simulink library "ammclib_bam_S32K3xx"  (R2016a)
(part 24 of 50)

      |       tmpOutCnt=tmpOutCnt+1;
      |       set_param([gcb '/fltState_Out'], 'Port', num2str(tmpOutCnt));
      |     end
      | 
      |   autoCalcEn=get_param(gcb,'autoCalcEn');
      |   if strcmp(autoCalcEn,'on')
      |     set_param(gcb,'MaskEnables',{'on','on','off','on','on','on','on','on','on','on','on','on','on','on','on','on','on','on','on','on','on','on','on','on','on','on','on','on','on','on','on','off'});
      |   else
      |     set_param(gcb,'MaskEnables',{'on','on','off','on','on','off','off','off','off','off','off','off','off','off','off','off','off','on','on','on','on','on','on','on','on','on','on','on','on','on','on','off'});
      |   end
      | 
      |     if (posblk(4) - posblk(2)) > 275
      |       height = 275;
      |       set_param(gcb,'Position',[posblk(1), posblk(2), posblk(3), posblk(2)+height])
      |     end
      |   end
      | else
      |   % shown state variables
      |   if strcmp(get_param([gcb '/fltUmaxDivImax'], 'BlockType'), 'Ground')
      |     posblk = get_param(gcb, 'Position');
      | 
      |     pos = get_param([gcb, '/fltUmaxDivImax'], 'Position');
      |     orient = get_param([gcb, '/fltUmaxDivImax'], 'Orientation');
      |     delete_block([gcb, '/fltUmaxDivImax']);
      |     add_block('built-in/Inport', [gcb, '/fltUmaxDivImax'], 'Position', pos, 'Orientation', orient, 'OutDataTypeStr', 'single');
      | 
      |     pos = get_param([gcb, '/fltLambdaW'], 'Position');
      |     orient = get_param([gcb, '/fltLambdaW'], 'Orientation');
      |     delete_block([gcb, '/fltLambdaW']);
      |     add_block('built-in/Inport', [gcb, '/fltLambdaW'], 'Position', pos, 'Orientation', orient, 'OutDataTypeStr', 'single');
      | 
      |     pos = get_param([gcb, '/fltLambdaFW'], 'Position');
      |     orient = get_param([gcb, '/fltLambdaFW'], 'Orientation');
      |     delete_block([gcb, '/fltLambdaFW']);
      |     add_block('built-in/Inport', [gcb, '/fltLambdaFW'], 'Position', pos, 'Orientation', orient, 'OutDataTypeStr', 'single');
      | 
      |     pos = get_param([gcb, '/fltPropGainQ'], 'Position');
      |     orient = get_param([gcb, '/fltPropGainQ'], 'Orientation');
      |     delete_block([gcb, '/fltPropGainQ']);
      |     add_block('built-in/Inport', [gcb, '/fltPropGainQ'], 'Position', pos, 'Orientation', orient, 'OutDataTypeStr', 'single');
      | 
      |     pos = get_param([gcb, '/fltIntegGainQ'], 'Position');
      |     orient = get_param([gcb, '/fltIntegGainQ'], 'Orientation');
      |     delete_block([gcb, '/fltIntegGainQ']);
      |     add_block('built-in/Inport', [gcb, '/fltIntegGainQ'], 'Position', pos, 'Orientation', orient, 'OutDataTypeStr', 'single');
      | 
      |     pos = get_param([gcb, '/fltLowerLimitQ'], 'Position');
      |     orient = get_param([gcb, '/fltLowerLimitQ'], 'Orientation');
      |     delete_block([gcb, '/fltLowerLimitQ']);
      |     add_block('built-in/Inport', [gcb, '/fltLowerLimitQ'], 'Position', pos, 'Orientation', orient, 'OutDataTypeStr', 'single');
      | 
      |     pos = get_param([gcb, '/fltUpperLimitQ'], 'Position');
      |     orient = get_param([gcb, '/fltUpperLimitQ'], 'Orientation');
      |     delete_block([gcb, '/fltUpperLimitQ']);
      |     add_block('built-in/Inport', [gcb, '/fltUpperLimitQ'], 'Position', pos, 'Orientation', orient, 'OutDataTypeStr', 'single');
      | 
      |     pos = get_param([gcb, '/fltPropGainFW'], 'Position');
      |     orient = get_param([gcb, '/fltPropGainFW'], 'Orientation');
      |     delete_block([gcb, '/fltPropGainFW']);
      |     add_block('built-in/Inport', [gcb, '/fltPropGainFW'], 'Position', pos, 'Orientation', orient, 'OutDataTypeStr', 'single');
      | 
      |     pos = get_param([gcb, '/fltIntegGainFW'], 'Position');
      |     orient = get_param([gcb, '/fltIntegGainFW'], 'Orientation');
      |     delete_block([gcb, '/fltIntegGainFW']);
      |     add_block('built-in/Inport', [gcb, '/fltIntegGainFW'], 'Position', pos, 'Orientation', orient, 'OutDataTypeStr', 'single');
      | 
      |     pos = get_param([gcb, '/fltLowerLimitFW'], 'Position');
      |     orient = get_param([gcb, '/fltLowerLimitFW'], 'Orientation');
      |     delete_block([gcb, '/fltLowerLimitFW']);
      |     add_block('built-in/Inport', [gcb, '/fltLowerLimitFW'], 'Position', pos, 'Orientation', orient, 'OutDataTypeStr', 'single');
      | 
      |     pos = get_param([gcb, '/fltUpperLimitFW'], 'Position');
      |     orient = get_param([gcb, '/fltUpperLimitFW'], 'Orientation');
      |     delete_block([gcb, '/fltUpperLimitFW']);
      |     add_block('built-in/Inport', [gcb, '/fltUpperLimitFW'], 'Position', pos, 'Orientation', orient, 'OutDataTypeStr', 'single');
      | 
      |     pos = get_param([gcb, '/fltRampUp'], 'Position');
      |     orient = get_param([gcb, '/fltRampUp'], 'Orientation');
      |     delete_block([gcb, '/fltRampUp']);
      |     add_block('built-in/Inport', [gcb, '/fltRampUp'], 'Position', pos, 'Orientation', orient, 'OutDataTypeStr', 'single');
      | 
      |     pos = get_param([gcb, '/fltRampDown'], 'Position');
      |     orient = get_param([gcb, '/fltRampDown'], 'Orientation');
      |     delete_block([gcb, '/fltRampDown']);
      |     add_block('built-in/Inport', [gcb, '/fltRampDown'], 'Position', pos, 'Orientation', orient, 'OutDataTypeStr', 'single');
      | 
      |     pos = get_param([gcb, '/fltIQReqK_1'], 'Position');
      |     orient = get_param([gcb, '/fltIQReqK_1'], 'Orientation');
      |     delete_block([gcb, '/fltIQReqK_1']);
      |     add_block('built-in/Inport', [gcb, '/fltIQReqK_1'], 'Position', pos, 'Orientation', orient, 'OutDataTypeStr', 'single');
      | 
      |     pos = get_param([gcb, '/fltAccW'], 'Position');
      |     orient = get_param([gcb, '/fltAccW'], 'Orientation');
      |     delete_block([gcb, '/fltAccW']);
      |     add_block('built-in/Inport', [gcb, '/fltAccW'], 'Position', pos, 'Orientation', orient, 'OutDataTypeStr', 'single');
      | 
      |     pos = get_param([gcb, '/fltAccFW'], 'Position');
      |     orient = get_param([gcb, '/fltAccFW'], 'Orientation');
      |     delete_block([gcb, '/fltAccFW']);
      |     add_block('built-in/Inport', [gcb, '/fltAccFW'], 'Position', pos, 'Orientation', orient, 'OutDataTypeStr', 'single');
      | 
      |     pos = get_param([gcb, '/fltIntegPartK_1Q'], 'Position');
      |     orient = get_param([gcb, '/fltIntegPartK_1Q'], 'Orientation');
      |     delete_block([gcb, '/fltIntegPartK_1Q']);
      |     add_block('built-in/Inport', [gcb, '/fltIntegPartK_1Q'], 'Position', pos, 'Orientation', orient, 'OutDataTypeStr', 'single');
      | 
      |     pos = get_param([gcb, '/fltInK_1Q'], 'Position');
      |     orient = get_param([gcb, '/fltInK_1Q'], 'Orientation');
      |     delete_block([gcb, '/fltInK_1Q']);
      |     add_block('built-in/Inport', [gcb, '/fltInK_1Q'], 'Position', pos, 'Orientation', orient, 'OutDataTypeStr', 'single');
      | 
      |     pos = get_param([gcb, '/fltIntegPartK_1FW'], 'Position');
      |     orient = get_param([gcb, '/fltIntegPartK_1FW'], 'Orientation');
      |     delete_block([gcb, '/fltIntegPartK_1FW']);
      |     add_block('built-in/Inport', [gcb, '/fltIntegPartK_1FW'], 'Position', pos, 'Orientation', orient, 'OutDataTypeStr', 'single');
      | 
      |     pos = get_param([gcb, '/fltInK_1FW'], 'Position');
      |     orient = get_param([gcb, '/fltInK_1FW'], 'Orientation');
      |     delete_block([gcb, '/fltInK_1FW']);
      |     add_block('built-in/Inport', [gcb, '/fltInK_1FW'], 'Position', pos, 'Orientation', orient, 'OutDataTypeStr', 'single');
      | 
      |     pos = get_param([gcb, '/fltState'], 'Position');
      |     orient = get_param([gcb, '/fltState'], 'Orientation');
      |     delete_block([gcb, '/fltState']);
      |     add_block('built-in/Inport', [gcb, '/fltState'], 'Position', pos, 'Orientation', orient, 'OutDataTypeStr', 'single');
      | 
      | 
      | 
      |     pos = get_param([gcb '/fltAccW_Out'], 'Position');
      |     orient = get_param([gcb '/fltAccW_Out'], 'Orientation');
      |     delete_block([gcb '/fltAccW_Out']);
      |     add_block('built-in/Outport', [gcb '/fltAccW_Out'], 'Position', pos, 'Orientation', orient);
      | 
      |     pos = get_param([gcb '/fltAccFW_Out'], 'Position');
      |     orient = get_param([gcb '/fltAccFW_Out'], 'Orientation');
      |     delete_block([gcb '/fltAccFW_Out']);
      |     add_block('built-in/Outport', [gcb '/fltAccFW_Out'], 'Position', pos, 'Orientation', orient);
      | 
      |     pos = get_param([gcb '/fltIntegPartK_1Q_Out'], 'Position');
      |     orient = get_param([gcb '/fltIntegPartK_1Q_Out'], 'Orientation');
      |     delete_block([gcb '/fltIntegPartK_1Q_Out']);
      |     add_block('built-in/Outport', [gcb '/fltIntegPartK_1Q_Out'], 'Position', pos, 'Orientation', orient);
      | 
      |     pos = get_param([gcb '/fltInK_1Q_Out'], 'Position');
      |     orient = get_param([gcb '/fltInK_1Q_Out'], 'Orientation');
      |     delete_block([gcb '/fltInK_1Q_Out']);
      |     add_block('built-in/Outport', [gcb '/fltInK_1Q_Out'], 'Position', pos, 'Orientation', orient);
      | 
      |     pos = get_param([gcb '/fltIntegPartK_1FW_Out'], 'Position');
      |     orient = get_param([gcb '/fltIntegPartK_1FW_Out'], 'Orientation');
      |     delete_block([gcb '/fltIntegPartK_1FW_Out']);
      |     add_block('built-in/Outport', [gcb '/fltIntegPartK_1FW_Out'], 'Position', pos, 'Orientation', orient);
      | 
      |     pos = get_param([gcb '/fltInK_1FW_Out'], 'Position');
      |     orient = get_param([gcb '/fltInK_1FW_Out'], 'Orientation');
      |     delete_block([gcb '/fltInK_1FW_Out']);
      |     add_block('built-in/Outport', [gcb '/fltInK_1FW_Out'], 'Position', pos, 'Orientation', orient);
      | 
      | 
      |     pmask=Simulink.Mask.get(gcb);
      |     pctrl=pmask.getParameter('SampleTime');
      |     pctrl.set('TypeOptions',{'fltVelocityReq/SampleTime','fltVelocityFbck/SampleTime','fltIQFbck/SampleTime','fltUQReq/SampleTime','fltUQLim/SampleTime','fltFilterMAWOut_preset/SampleTime','fltFilterMAFWOut_preset/SampleTime','fltControllerPIpAWQOut_preset/SampleTime','fltControllerPIpAWFWOut_preset/SampleTime','fltRampOut_preset/SampleTime','fltUmaxDivImax/SampleTime','fltLambdaW/SampleTime','fltLambdaFW/SampleTime','fltPropGainQ/SampleTime','fltIntegGainQ/SampleTime','fltLowerLimitQ/SampleTime','fltUpperLimitQ/SampleTime','fltPropGainFW/SampleTime','fltIntegGainFW/SampleTime','fltLowerLimitFW/SampleTime','fltUpperLimitFW/SampleTime','fltRampUp/SampleTime','fltRampDown/SampleTime','fltIQReqK_1/SampleTime','fltAccW/SampleTime','fltAccFW/SampleTime','fltIntegPartK_1Q/SampleTime','fltInK_1Q/SampleTime','fltIntegPartK_1FW/SampleTime','fltInK_1FW/SampleTime','fltState/SampleTime'});
      | 
      |     if (showDebugOutputs == 2) && (strcmp(get_param([gcb '/fltWReqFilt'], 'BlockType'), 'Terminator'))
      |       pos = get_param([gcb '/fltWReqFilt'], 'Position');
      |       orient = get_param([gcb '/fltWReqFilt'], 'Orientation');
      |       delete_block([gcb '/fltWReqFilt']);
      |       add_block('built-in/Outport', [gcb '/fltWReqFilt'], 'Position', pos, 'Orientation', orient);
      | 
      |       pos = get_param([gcb '/fltWErr'], 'Position');
      |       orient = get_param([gcb '/fltWErr'], 'Orientation');
      |       delete_block([gcb '/fltWErr']);
      |       add_block('built-in/Outport', [gcb '/fltWErr'], 'Position', pos, 'Orientation', orient);
      | 
      |       pos = get_param([gcb '/fltIDQReqAmp'], 'Position');
      |       orient = get_param([gcb '/fltIDQReqAmp'], 'Orientation');
      |       delete_block([gcb '/fltIDQReqAmp']);
      |       add_block('built-in/Outport', [gcb '/fltIDQReqAmp'], 'Position', pos, 'Orientation', orient);
      | 
      |       pos = get_param([gcb '/fltWFbckFilt'], 'Position');
      |       orient = get_param([gcb '/fltWFbckFilt'], 'Orientation');
      |       delete_block([gcb '/fltWFbckFilt']);
      |       add_block('built-in/Outport', [gcb '/fltWFbckFilt'], 'Position', pos, 'Orientation', orient);
      | 
      |       pos = get_param([gcb '/fltIQErrSign'], 'Position');
      |       orient = get_param([gcb '/fltIQErrSign'], 'Orientation');
      |       delete_block([gcb '/fltIQErrSign']);
      |       add_block('built-in/Outport', [gcb '/fltIQErrSign'], 'Position', pos, 'Orientation', orient);
      | 
      |       pos = get_param([gcb '/fltFWErr'], 'Position');
      |       orient = get_param([gcb '/fltFWErr'], 'Orientation');
      |       delete_block([gcb '/fltFWErr']);
      |       add_block('built-in/Outport', [gcb '/fltFWErr'], 'Position', pos, 'Orientation', orient);
      | 
      |       pos = get_param([gcb '/fltIQErr'], 'Position');
      |       orient = get_param([gcb '/fltIQErr'], 'Orientation');
      |       delete_block([gcb '/fltIQErr']);
      |       add_block('built-in/Outport', [gcb '/fltIQErr'], 'Position', pos, 'Orientation', orient);
      | 
      |       pos = get_param([gcb '/fltUQErr'], 'Position');
      |       orient = get_param([gcb '/fltUQErr'], 'Orientation');
      |       delete_block([gcb '/fltUQErr']);
      |       add_block('built-in/Outport', [gcb '/fltUQErr'], 'Position', pos, 'Orientation', orient);
      | 
      |       pos = get_param([gcb '/fltFWErrFilt'], 'Position');
      |       orient = get_param([gcb '/fltFWErrFilt'], 'Orientation');
      |       delete_block([gcb '/fltFWErrFilt']);
      |       add_block('built-in/Outport', [gcb '/fltFWErrFilt'], 'Position', pos, 'Orientation', orient);
      | 
      |       pos = get_param([gcb '/fltFWAngle'], 'Position');
      |       orient = get_param([gcb '/fltFWAngle'], 'Orientation');
      |       delete_block([gcb '/fltFWAngle']);
      |       add_block('built-in/Outport', [gcb '/fltFWAngle'], 'Position', pos, 'Orientation', orient);
      | 
      |       pos = get_param([gcb '/fltFWSin'], 'Position');
      |       orient = get_param([gcb '/fltFWSin'], 'Orientation');
      |       delete_block([gcb '/fltFWSin']);
      |       add_block('built-in/Outport', [gcb '/fltFWSin'], 'Position', pos, 'Orientation', orient);
      | 
      |       pos = get_param([gcb '/fltFWCos'], 'Position');
      |       orient = get_param([gcb '/fltFWCos'], 'Orientation');
      |       delete_block([gcb '/fltFWCos']);
      |       add_block('built-in/Outport', [gcb '/fltFWCos'], 'Position', pos, 'Orientation', orient);
      | 
      |     end
      | 
      |     set_param([gcb '/fltVelocityReq'], 'Port', '1');
      |     set_param([gcb '/fltVelocityFbck'], 'Port', '2');
      |     set_param([gcb '/fltIQFbck'], 'Port', '3');
      |     set_param([gcb '/fltUQReq'], 'Port', '4');
      |     set_param([gcb '/fltUQLim'], 'Port', '5');
      |     set_param([gcb '/fltFilterMAWOut_preset'], 'Port', '6');
      |     set_param([gcb '/fltFilterMAFWOut_preset'], 'Port', '7');
      |     set_param([gcb '/fltControllerPIpAWQOut_preset'], 'Port', '8');
      |     set_param([gcb '/fltControllerPIpAWFWOut_preset'], 'Port', '9');
      |     set_param([gcb '/fltRampOut_preset'], 'Port', '10');
      |     set_param([gcb '/fltUmaxDivImax'], 'Port', '11');
      |     set_param([gcb '/fltLambdaW'], 'Port', '12');
      |     set_param([gcb '/fltLambdaFW'], 'Port', '13');
      |     set_param([gcb '/fltPropGainQ'], 'Port', '14');
      |     set_param([gcb '/fltIntegGainQ'], 'Port', '15');
      |     set_param([gcb '/fltLowerLimitQ'], 'Port', '16');
      |     set_param([gcb '/fltUpperLimitQ'], 'Port', '17');
      |     set_param([gcb '/fltPropGainFW'], 'Port', '18');
      |     set_param([gcb '/fltIntegGainFW'], 'Port', '19');
      |     set_param([gcb '/fltLowerLimitFW'], 'Port', '20');
      |     set_param([gcb '/fltUpperLimitFW'], 'Port', '21');
      |     set_param([gcb '/fltRampUp'], 'Port', '22');
      |     set_param([gcb '/fltRampDown'], 'Port', '23');
      |     set_param([gcb '/fltIQReqK_1'], 'Port', '24');
      |     set_param([gcb '/fltAccW'], 'Port', '25');
      |     set_param([gcb '/fltAccFW'], 'Port', '26');
      |     set_param([gcb '/fltIntegPartK_1Q'], 'Port', '27');
      |     set_param([gcb '/fltInK_1Q'], 'Port', '28');
      |     set_param([gcb '/fltIntegPartK_1FW'], 'Port', '29');
      |     set_param([gcb '/fltInK_1FW'], 'Port', '30');
      |     set_param([gcb '/fltState'], 'Port', '31');
      | 
      |     if (showDebugOutputs == 2)
      |       tmpOutCnt=0;
      |       tmpOutCnt=tmpOutCnt+1;
      |       set_param([gcb '/pIDQReq'], 'Port', num2str(tmpOutCnt));
      |       tmpOutCnt=tmpOutCnt+1;
      |       set_param([gcb '/u16LimitFlagQ'], 'Port', num2str(tmpOutCnt));
      |       tmpOutCnt=tmpOutCnt+1;
      |       set_param([gcb '/u16LimitFlagFW'], 'Port', num2str(tmpOutCnt));
      |       tmpOutCnt=tmpOutCnt+1;
      |       set_param([gcb '/fltWReqFilt'], 'Port', num2str(tmpOutCnt));
      |       tmpOutCnt=tmpOutCnt+1;
      |       set_param([gcb '/fltWErr'], 'Port', num2str(tmpOutCnt));
      |       tmpOutCnt=tmpOutCnt+1;
      |       set_param([gcb '/fltIDQReqAmp'], 'Port', num2str(tmpOutCnt));
      |       tmpOutCnt=tmpOutCnt+1;
      |       set_param([gcb '/fltWFbckFilt'], 'Port', num2str(tmpOutCnt));
      |       tmpOutCnt=tmpOutCnt+1;
      |       set_param([gcb '/fltIQErrSign'], 'Port', num2str(tmpOutCnt));
      |       tmpOutCnt=tmpOutCnt+1;
      |       set_param([gcb '/fltFWErr'], 'Port', num2str(tmpOutCnt));
      |       tmpOutCnt=tmpOutCnt+1;
      |       set_param([gcb '/fltIQErr'], 'Port', num2str(tmpOutCnt));
      |       tmpOutCnt=tmpOutCnt+1;
      |       set_param([gcb '/fltUQErr'], 'Port', num2str(tmpOutCnt));
      |       tmpOutCnt=tmpOutCnt+1;
      |       set_param([gcb '/fltFWErrFilt'], 'Port', num2str(tmpOutCnt));
      |       tmpOutCnt=tmpOutCnt+1;
      |       set_param([gcb '/fltFWAngle'], 'Port', num2str(tmpOutCnt));
      |       tmpOutCnt=tmpOutCnt+1;
      |       set_param([gcb '/fltFWSin'], 'Port', num2str(tmpOutCnt));
      |       tmpOutCnt=tmpOutCnt+1;
      |       set_param([gcb '/fltFWCos'], 'Port', num2str(tmpOutCnt));
      |       tmpOutCnt=tmpOutCnt+1;
      |       set_param([gcb '/fltAccW_Out'], 'Port', num2str(tmpOutCnt));
      |       tmpOutCnt=tmpOutCnt+1;
      |       set_param([gcb '/fltAccFW_Out'], 'Port', num2str(tmpOutCnt));
      |       tmpOutCnt=tmpOutCnt+1;
      |       set_param([gcb '/fltIntegPartK_1Q_Out'], 'Port', num2str(tmpOutCnt));
      |       tmpOutCnt=tmpOutCnt+1;
      |       set_param([gcb '/fltInK_1Q_Out'], 'Port', num2str(tmpOutCnt));
      |       tmpOutCnt=tmpOutCnt+1;
      |       set_param([gcb '/fltIntegPartK_1FW_Out'], 'Port', num2str(tmpOutCnt));
      |       tmpOutCnt=tmpOutCnt+1;
      |       set_param([gcb '/fltInK_1FW_Out'], 'Port', num2str(tmpOutCnt));
      |       if strcmp(get_param([gcb '/fltState_Out'], 'BlockType'), 'Outport')
      |         tmpOutCnt=tmpOutCnt+1;
      |         set_param([gcb '/fltState_Out'], 'Port', num2str(tmpOutCnt));
      |       end
      |     else
      |       tmpOutCnt=0;
      |       tmpOutCnt=tmpOutCnt+1;
      |       set_param([gcb '/pIDQReq'], 'Port', num2str(tmpOutCnt));
      |       tmpOutCnt=tmpOutCnt+1;
      |       set_param([gcb '/u16LimitFlagQ'], 'Port', num2str(tmpOutCnt));
      |       tmpOutCnt=tmpOutCnt+1;
      |       set_param([gcb '/u16LimitFlagFW'], 'Port', num2str(tmpOutCnt));
      |       tmpOutCnt=tmpOutCnt+1;
      |       set_param([gcb '/fltAccW_Out'], 'Port', num2str(tmpOutCnt));
      |       tmpOutCnt=tmpOutCnt+1;
      |       set_param([gcb '/fltAccFW_Out'], 'Port', num2str(tmpOutCnt));
      |       tmpOutCnt=tmpOutCnt+1;
      |       set_param([gcb '/fltIntegPartK_1Q_Out'], 'Port', num2str(tmpOutCnt));
      |       tmpOutCnt=tmpOutCnt+1;
      |       set_param([gcb '/fltInK_1Q_Out'], 'Port', num2str(tmpOutCnt));
      |       tmpOutCnt=tmpOutCnt+1;
      |       set_param([gcb '/fltIntegPartK_1FW_Out'], 'Port', num2str(tmpOutCnt));
      |       tmpOutCnt=tmpOutCnt+1;
      |       set_param([gcb '/fltInK_1FW_Out'], 'Port', num2str(tmpOutCnt));
      |       if strcmp(get_param([gcb '/fltState_Out'], 'BlockType'), 'Outport')
      |         tmpOutCnt=tmpOutCnt+1;
      |         set_param([gcb '/fltState_Out'], 'Port', num2str(tmpOutCnt));
      |       end
      |     end
      | 
      |     set_param(gcb,'MaskEnables',{'on','on','on','on','on','off','off','off','off','off','off','off','off','off','off','off','off','off','off','off','off','off','off','off','off','off','off','off','off','off','off','off'});
      | 
      |     if (posblk(4) - posblk(2)) < 800
      |       height = 800;
      |       set_param(gcb,'Position',[posblk(1), posblk(2), posblk(3), posblk(2)+height])
      |     end
      |   else
      |     if (showDebugOutputs == 2) && (strcmp(get_param([gcb '/fltWReqFilt'], 'BlockType'), 'Terminator'))
      |       % shown debugging outputs
      |       pos = get_param([gcb '/fltWReqFilt'], 'Position');
      |       orient = get_param([gcb '/fltWReqFilt'], 'Orientation');
      |       delete_block([gcb '/fltWReqFilt']);
      |       add_block('built-in/Outport', [gcb '/fltWReqFilt'], 'Position', pos, 'Orientation', orient);
      | 
      |       pos = get_param([gcb '/fltWErr'], 'Position');
      |       orient = get_param([gcb '/fltWErr'], 'Orientation');
      |       delete_block([gcb '/fltWErr']);
      |       add_block('built-in/Outport', [gcb '/fltWErr'], 'Position', pos, 'Orientation', orient);
      | 
      |       pos = get_param([gcb '/fltIDQReqAmp'], 'Position');
      |       orient = get_param([gcb '/fltIDQReqAmp'], 'Orientation');
      |       delete_block([gcb '/fltIDQReqAmp']);
      |       add_block('built-in/Outport', [gcb '/fltIDQReqAmp'], 'Position', pos, 'Orientation', orient);
      | 
      |       pos = get_param([gcb '/fltWFbckFilt'], 'Position');
      |       orient = get_param([gcb '/fltWFbckFilt'], 'Orientation');
      |       delete_block([gcb '/fltWFbckFilt']);
      |       add_block('built-in/Outport', [gcb '/fltWFbckFilt'], 'Position', pos, 'Orientation', orient);
      | 
      |       pos = get_param([gcb '/fltIQErrSign'], 'Position');
      |       orient = get_param([gcb '/fltIQErrSign'], 'Orientation');
      |       delete_block([gcb '/fltIQErrSign']);
      |       add_block('built-in/Outport', [gcb '/fltIQErrSign'], 'Position', pos, 'Orientation', orient);
      | 
      |       pos = get_param([gcb '/fltFWErr'], 'Position');
      |       orient = get_param([gcb '/fltFWErr'], 'Orientation');
      |       delete_block([gcb '/fltFWErr']);
      |       add_block('built-in/Outport', [gcb '/fltFWErr'], 'Position', pos, 'Orientation', orient);
      | 
      |       pos = get_param([gcb '/fltIQErr'], 'Position');
      |       orient = get_param([gcb '/fltIQErr'], 'Orientation');
      |       delete_block([gcb '/fltIQErr']);
      |       add_block('built-in/Outport', [gcb '/fltIQErr'], 'Position', pos, 'Orientation', orient);
      | 
      |       pos = get_param([gcb '/fltUQErr'], 'Position');
      |       orient = get_param([gcb '/fltUQErr'], 'Orientation');
      |       delete_block([gcb '/fltUQErr']);
      |       add_block('built-in/Outport', [gcb '/fltUQErr'], 'Position', pos, 'Orientation', orient);
      | 
      |       pos = get_param([gcb '/fltFWErrFilt'], 'Position');
      |       orient = get_param([gcb '/fltFWErrFilt'], 'Orientation');
      |       delete_block([gcb '/fltFWErrFilt']);
      |       add_block('built-in/Outport', [gcb '/fltFWErrFilt'], 'Position', pos, 'Orientation', orient);
      | 
      |       pos = get_param([gcb '/fltFWAngle'], 'Position');
      |       orient = get_param([gcb '/fltFWAngle'], 'Orientation');
      |       delete_block([gcb '/fltFWAngle']);
      |       add_block('built-in/Outport', [gcb '/fltFWAngle'], 'Position', pos, 'Orientation', orient);
      | 
      |       pos = get_param([gcb '/fltFWSin'], 'Position');
      |       orient = get_param([gcb '/fltFWSin'], 'Orientation');
      |       delete_block([gcb '/fltFWSin']);
      |       add_block('built-in/Outport', [gcb '/fltFWSin'], 'Position', pos, 'Orientation', orient);
      | 
      |       pos = get_param([gcb '/fltFWCos'], 'Position');
      |       orient = get_param([gcb '/fltFWCos'], 'Orientation');
      |       delete_block([gcb '/fltFWCos']);
      |       add_block('built-in/Outport', [gcb '/fltFWCos'], 'Position', pos, 'Orientation', orient);
      | 
      |       tmpOutCnt=0;
      |       tmpOutCnt=tmpOutCnt+1;
      |       set_param([gcb '/pIDQReq'], 'Port', num2str(tmpOutCnt));
      |       tmpOutCnt=tmpOutCnt+1;
      |       set_param([gcb '/u16LimitFlagQ'], 'Port', num2str(tmpOutCnt));
      |       tmpOutCnt=tmpOutCnt+1;
      |       set_param([gcb '/u16LimitFlagFW'], 'Port', num2str(tmpOutCnt));
      |       tmpOutCnt=tmpOutCnt+1;
      |       set_param([gcb '/fltWReqFilt'], 'Port', num2str(tmpOutCnt));
      |       tmpOutCnt=tmpOutCnt+1;
      |       set_param([gcb '/fltWErr'], 'Port', num2str(tmpOutCnt));
      |       tmpOutCnt=tmpOutCnt+1;
      |       set_param([gcb '/fltIDQReqAmp'], 'Port', num2str(tmpOutCnt));
      |       tmpOutCnt=tmpOutCnt+1;
      |       set_param([gcb '/fltWFbckFilt'], 'Port', num2str(tmpOutCnt));
      |       tmpOutCnt=tmpOutCnt+1;
      |       set_param([gcb '/fltIQErrSign'], 'Port', num2str(tmpOutCnt));
      |       tmpOutCnt=tmpOutCnt+1;
      |       set_param([gcb '/fltFWErr'], 'Port', num2str(tmpOutCnt));
      |       tmpOutCnt=tmpOutCnt+1;
      |       set_param([gcb '/fltIQErr'], 'Port', num2str(tmpOutCnt));
      |       tmpOutCnt=tmpOutCnt+1;
      |       set_param([gcb '/fltUQErr'], 'Port', num2str(tmpOutCnt));
      |       tmpOutCnt=tmpOutCnt+1;
      |       set_param([gcb '/fltFWErrFilt'], 'Port', num2str(tmpOutCnt));
      |       tmpOutCnt=tmpOutCnt+1;
      |       set_param([gcb '/fltFWAngle'], 'Port', num2str(tmpOutCnt));
      |       tmpOutCnt=tmpOutCnt+1;
      |       set_param([gcb '/fltFWSin'], 'Port', num2str(tmpOutCnt));
      |       tmpOutCnt=tmpOutCnt+1;
      |       set_param([gcb '/fltFWCos'], 'Port', num2str(tmpOutCnt));
      |       tmpOutCnt=tmpOutCnt+1;
      |       set_param([gcb '/fltAccW_Out'], 'Port', num2str(tmpOutCnt));
      |       tmpOutCnt=tmpOutCnt+1;
      |       set_param([gcb '/fltAccFW_Out'], 'Port', num2str(tmpOutCnt));
      |       tmpOutCnt=tmpOutCnt+1;
      |       set_param([gcb '/fltIntegPartK_1Q_Out'], 'Port', num2str(tmpOutCnt));
      |       tmpOutCnt=tmpOutCnt+1;
      |       set_param([gcb '/fltInK_1Q_Out'], 'Port', num2str(tmpOutCnt));
      |       tmpOutCnt=tmpOutCnt+1;
      |       set_param([gcb '/fltIntegPartK_1FW_Out'], 'Port', num2str(tmpOutCnt));
      |       tmpOutCnt=tmpOutCnt+1;
      |       set_param([gcb '/fltInK_1FW_Out'], 'Port', num2str(tmpOutCnt));
      |       if strcmp(get_param([gcb '/fltState_Out'], 'BlockType'), 'Outport')
      |         tmpOutCnt=tmpOutCnt+1;
      |         set_param([gcb '/fltState_Out'], 'Port', num2str(tmpOutCnt));
      |       end
      |     elseif (showDebugOutputs == 1) && (strcmp(get_param([gcb '/fltWReqFilt'], 'BlockType'), 'Outport'))
      |       % hidden debugging outputs
      |       pos = get_param([gcb '/fltWReqFilt'], 'Position');
      |       orient = get_param([gcb '/fltWReqFilt'], 'Orientation');
      |       delete_block([gcb '/fltWReqFilt']);
      |       add_block('built-in/Terminator', [gcb '/fltWReqFilt'], 'Position', pos, 'Orientation', orient);
      | 
      |       pos = get_param([gcb '/fltWErr'], 'Position');
      |       orient = get_param([gcb '/fltWErr'], 'Orientation');
      |       delete_block([gcb '/fltWErr']);
      |       add_block('built-in/Terminator', [gcb '/fltWErr'], 'Position', pos, 'Orientation', orient);
      | 
      |       pos = get_param([gcb '/fltIDQReqAmp'], 'Position');
      |       orient = get_param([gcb '/fltIDQReqAmp'], 'Orientation');
      |       delete_block([gcb '/fltIDQReqAmp']);
      |       add_block('built-in/Terminator', [gcb '/fltIDQReqAmp'], 'Position', pos, 'Orientation', orient);
      | 
      |       pos = get_param([gcb '/fltWFbckFilt'], 'Position');
      |       orient = get_param([gcb '/fltWFbckFilt'], 'Orientation');
      |       delete_block([gcb '/fltWFbckFilt']);
      |       add_block('built-in/Terminator', [gcb '/fltWFbckFilt'], 'Position', pos, 'Orientation', orient);
      | 
      |       pos = get_param([gcb '/fltIQErrSign'], 'Position');
      |       orient = get_param([gcb '/fltIQErrSign'], 'Orientation');
      |       delete_block([gcb '/fltIQErrSign']);
      |       add_block('built-in/Terminator', [gcb '/fltIQErrSign'], 'Position', pos, 'Orientation', orient);
      | 
      |       pos = get_param([gcb '/fltFWErr'], 'Position');
      |       orient = get_param([gcb '/fltFWErr'], 'Orientation');
      |       delete_block([gcb '/fltFWErr']);
      |       add_block('built-in/Terminator', [gcb '/fltFWErr'], 'Position', pos, 'Orientation', orient);
      | 
      |       pos = get_param([gcb '/fltIQErr'], 'Position');
      |       orient = get_param([gcb '/fltIQErr'], 'Orientation');
      |       delete_block([gcb '/fltIQErr']);
      |       add_block('built-in/Terminator', [gcb '/fltIQErr'], 'Position', pos, 'Orientation', orient);
      | 
      |       pos = get_param([gcb '/fltUQErr'], 'Position');
      |       orient = get_param([gcb '/fltUQErr'], 'Orientation');
      |       delete_block([gcb '/fltUQErr']);
      |       add_block('built-in/Terminator', [gcb '/fltUQErr'], 'Position', pos, 'Orientation', orient);
      | 
      |       pos = get_param([gcb '/fltFWErrFilt'], 'Position');
      |       orient = get_param([gcb '/fltFWErrFilt'], 'Orientation');
      |       delete_block([gcb '/fltFWErrFilt']);
      |       add_block('built-in/Terminator', [gcb '/fltFWErrFilt'], 'Position', pos, 'Orientation', orient);
      | 
      |       pos = get_param([gcb '/fltFWAngle'], 'Position');
      |       orient = get_param([gcb '/fltFWAngle'], 'Orientation');
      |       delete_block([gcb '/fltFWAngle']);
      |       add_block('built-in/Terminator', [gcb '/fltFWAngle'], 'Position', pos, 'Orientation', orient);
      | 
      |       pos = get_param([gcb '/fltFWSin'], 'Position');
      |       orient = get_param([gcb '/fltFWSin'], 'Orientation');
      |       delete_block([gcb '/fltFWSin']);
      |       add_block('built-in/Terminator', [gcb '/fltFWSin'], 'Position', pos, 'Orientation', orient);
      | 
      |       pos = get_param([gcb '/fltFWCos'], 'Position');
      |       orient = get_param([gcb '/fltFWCos'], 'Orientation');
      |       delete_block([gcb '/fltFWCos']);
      |       add_block('built-in/Terminator', [gcb '/fltFWCos'], 'Position', pos, 'Orientation', orient);
      | 
      |       tmpOutCnt=0;
      |       tmpOutCnt=tmpOutCnt+1;
      |       set_param([gcb '/pIDQReq'], 'Port', num2str(tmpOutCnt));
      |       tmpOutCnt=tmpOutCnt+1;
      |       set_param([gcb '/u16LimitFlagQ'], 'Port', num2str(tmpOutCnt));
      |       tmpOutCnt=tmpOutCnt+1;
      |       set_param([gcb '/u16LimitFlagFW'], 'Port', num2str(tmpOutCnt));
      |       tmpOutCnt=tmpOutCnt+1;
      |       set_param([gcb '/fltAccW_Out'], 'Port', num2str(tmpOutCnt));
      |       tmpOutCnt=tmpOutCnt+1;
      |       set_param([gcb '/fltAccFW_Out'], 'Port', num2str(tmpOutCnt));
      |       tmpOutCnt=tmpOutCnt+1;
      |       set_param([gcb '/fltIntegPartK_1Q_Out'], 'Port', num2str(tmpOutCnt));
      |       tmpOutCnt=tmpOutCnt+1;
      |       set_param([gcb '/fltInK_1Q_Out'], 'Port', num2str(tmpOutCnt));
      |       tmpOutCnt=tmpOutCnt+1;
      |       set_param([gcb '/fltIntegPartK_1FW_Out'], 'Port', num2str(tmpOutCnt));
      |       tmpOutCnt=tmpOutCnt+1;
      |       set_param([gcb '/fltInK_1FW_Out'], 'Port', num2str(tmpOutCnt));
      |       if strcmp(get_param([gcb '/fltState_Out'], 'BlockType'), 'Outport')
      |         tmpOutCnt=tmpOutCnt+1;
      |         set_param([gcb '/fltState_Out'], 'Port', num2str(tmpOutCnt));
      |       end
      |     end
      |   end
      | end
      | if strcmp(get_param(gcb,'fltState_Out_showOutput'),'on')
      |   if strcmp(get_param([gcb '/fltState_Out'], 'BlockType'), 'Terminator')
      |     pos = get_param([gcb '/fltState_Out'], 'Position');
      |     orient = get_param([gcb '/fltState_Out'], 'Orientation');
      |     delete_block([gcb '/fltState_Out']);
      |     add_block('built-in/Outport', [gcb '/fltState_Out'], 'Position', pos, 'Orientation', orient);
      |     outputsChanged = 1;
      |   end
      | else
      |   if strcmp(get_param([gcb '/fltState_Out'], 'BlockType'), 'Outport')
      |     pos = get_param([gcb '/fltState_Out'], 'Position');
      |     orient = get_param([gcb '/fltState_Out'], 'Orientation');
      |     delete_block([gcb '/fltState_Out']);
      |     add_block('built-in/Terminator', [gcb '/fltState_Out'], 'Position', pos, 'Orientation', orient);
      |     outputsChanged = 1;
      |   end
      | end
      | if outputsChanged == 1;
      |   tmpOutCnt = 0;
      |   if strcmp(get_param([gcb '/pIDQReq'], 'BlockType'), 'Outport')
      |     tmpOutCnt = tmpOutCnt + 1;
      |     set_param([gcb '/pIDQReq'], 'Port', num2str(tmpOutCnt));
      |   end
      |   if strcmp(get_param([gcb '/u16LimitFlagQ'], 'BlockType'), 'Outport')
      |     tmpOutCnt = tmpOutCnt + 1;
      |     set_param([gcb '/u16LimitFlagQ'], 'Port', num2str(tmpOutCnt));
      |   end
      |   if strcmp(get_param([gcb '/u16LimitFlagFW'], 'BlockType'), 'Outport')
      |     tmpOutCnt = tmpOutCnt + 1;
      |     set_param([gcb '/u16LimitFlagFW'], 'Port', num2str(tmpOutCnt));
      |   end
      |   if strcmp(get_param([gcb '/fltWReqFilt'], 'BlockType'), 'Outport')
      |     tmpOutCnt = tmpOutCnt + 1;
      |     set_param([gcb '/fltWReqFilt'], 'Port', num2str(tmpOutCnt));
      |   end
      |   if strcmp(get_param([gcb '/fltWErr'], 'BlockType'), 'Outport')
      |     tmpOutCnt = tmpOutCnt + 1;
      |     set_param([gcb '/fltWErr'], 'Port', num2str(tmpOutCnt));
      |   end
      |   if strcmp(get_param([gcb '/fltIDQReqAmp'], 'BlockType'), 'Outport')
      |     tmpOutCnt = tmpOutCnt + 1;
      |     set_param([gcb '/fltIDQReqAmp'], 'Port', num2str(tmpOutCnt));
      |   end
      |   if strcmp(get_param([gcb '/fltWFbckFilt'], 'BlockType'), 'Outport')
      |     tmpOutCnt = tmpOutCnt + 1;
      |     set_param([gcb '/fltWFbckFilt'], 'Port', num2str(tmpOutCnt));
      |   end
      |   if strcmp(get_param([gcb '/fltIQErrSign'], 'BlockType'), 'Outport')
      |     tmpOutCnt = tmpOutCnt + 1;
      |     set_param([gcb '/fltIQErrSign'], 'Port', num2str(tmpOutCnt));
      |   end
      |   if strcmp(get_param([gcb '/fltFWErr'], 'BlockType'), 'Outport')
      |     tmpOutCnt = tmpOutCnt + 1;
      |     set_param([gcb '/fltFWErr'], 'Port', num2str(tmpOutCnt));
      |   end
      |   if strcmp(get_param([gcb '/fltIQErr'], 'BlockType'), 'Outport')
      |     tmpOutCnt = tmpOutCnt + 1;
      |     set_param([gcb '/fltIQErr'], 'Port', num2str(tmpOutCnt));
      |   end
      |   if strcmp(get_param([gcb '/fltUQErr'], 'BlockType'), 'Outport')
      |     tmpOutCnt = tmpOutCnt + 1;
      |     set_param([gcb '/fltUQErr'], 'Port', num2str(tmpOutCnt));
      |   end
      |   if strcmp(get_param([gcb '/fltFWErrFilt'], 'BlockType'), 'Outport')
      |     tmpOutCnt = tmpOutCnt + 1;
      |     set_param([gcb '/fltFWErrFilt'], 'Port', num2str(tmpOutCnt));
      |   end
      |   if strcmp(get_param([gcb '/fltFWAngle'], 'BlockType'), 'Outport')
      |     tmpOutCnt = tmpOutCnt + 1;
      |     set_param([gcb '/fltFWAngle'], 'Port', num2str(tmpOutCnt));
      |   end
      |   if strcmp(get_param([gcb '/fltFWSin'], 'BlockType'), 'Outport')
      |     tmpOutCnt = tmpOutCnt + 1;
      |     set_param([gcb '/fltFWSin'], 'Port', num2str(tmpOutCnt));
      |   end
      |   if strcmp(get_param([gcb '/fltFWCos'], 'BlockType'), 'Outport')
      |     tmpOutCnt = tmpOutCnt + 1;
      |     set_param([gcb '/fltFWCos'], 'Port', num2str(tmpOutCnt));
      |   end
      |   if strcmp(get_param([gcb '/fltAccW_Out'], 'BlockType'), 'Outport')
      |     tmpOutCnt = tmpOutCnt + 1;
      |     set_param([gcb '/fltAccW_Out'], 'Port', num2str(tmpOutCnt));
      |   end
      |   if strcmp(get_param([gcb '/fltAccFW_Out'], 'BlockType'), 'Outport')
      |     tmpOutCnt = tmpOutCnt + 1;
      |     set_param([gcb '/fltAccFW_Out'], 'Port', num2str(tmpOutCnt));
      |   end
      |   if strcmp(get_param([gcb '/fltIntegPartK_1Q_Out'], 'BlockType'), 'Outport')
      |     tmpOutCnt = tmpOutCnt + 1;
      |     set_param([gcb '/fltIntegPartK_1Q_Out'], 'Port', num2str(tmpOutCnt));
      |   end
      |   if strcmp(get_param([gcb '/fltInK_1Q_Out'], 'BlockType'), 'Outport')
      |     tmpOutCnt = tmpOutCnt + 1;
      |     set_param([gcb '/fltInK_1Q_Out'], 'Port', num2str(tmpOutCnt));
      |   end
      |   if strcmp(get_param([gcb '/fltIntegPartK_1FW_Out'], 'BlockType'), 'Outport')
      |     tmpOutCnt = tmpOutCnt + 1;
      |     set_param([gcb '/fltIntegPartK_1FW_Out'], 'Port', num2str(tmpOutCnt));
      |   end
      |   if strcmp(get_param([gcb '/fltInK_1FW_Out'], 'BlockType'), 'Outport')
      |     tmpOutCnt = tmpOutCnt + 1;
      |     set_param([gcb '/fltInK_1FW_Out'], 'Port', num2str(tmpOutCnt));
      |   end
      |   if strcmp(get_param([gcb '/fltState_Out'], 'BlockType'), 'Outport')
      |     tmpOutCnt = tmpOutCnt + 1;
      |     set_param([gcb '/fltState_Out'], 'Port', num2str(tmpOutCnt));
      |   end
      | end
      settings: RTWSystemCode=Inline
      mask Help: web([fileparts(which('ammclib_bam_S32K3xx.slx')) '/../doc/S32K3XXMCLUG.pdf'], '-browser')
      mask TypeOptions showStates: Hide (faster execution) | Show (allows debugging; connect feedback loops manually)
      mask Callback showStates:
      | maskStr=get_param(gcb,'showStates');
      | if strcmp(maskStr,'Hide (faster execution)')
      |   autoCalcEn=get_param(gcb,'autoCalcEn');
      |   if strcmp(autoCalcEn,'on')
      |     set_param(gcb,'MaskEnables',{'on','on','off','on','on','on','on','on','on','on','on','on','on','on','on','on','on','on','on','on','on','on','on','on','on','on','on','on','on','on','on','off'});
      |   else
      |     set_param(gcb,'MaskEnables',{'on','on','off','on','on','off','off','off','off','off','off','off','off','off','off','off','off','on','on','on','on','on','on','on','on','on','on','on','on','on','on','off'});
      |   end
      | else
      |   set_param(gcb,'MaskEnables',{'on','on','on','on','on','off','off','off','off','off','off','off','off','off','off','off','off','off','off','off','off','off','off','off','off','off','off','off','off','off','off','off'});
      | end
      mask TypeOptions resetStatesEnable: Pre-set according to the first set of inputs after reset | Clear to zero
      mask TypeOptions showDebugOutputs: Hide | Show
      mask TypeOptions SampleTime: fltVelocityReq/SampleTime | fltVelocityFbck/SampleTime | fltIQFbck/SampleTime | fltUQReq/SampleTime | fltUQLim/SampleTime | fltFilterMAWOut_preset/SampleTime | fltFilterMAFWOut_preset/SampleTime | fltControllerPIpAWQOut_preset/SampleTime | fltControllerPIpAWFWOut_preset/SampleTime | fltRampOut_preset/SampleTime
      mask Callback SampleTime:
      | p=Simulink.Mask.get(gcb);
      | hintText=p.getDialogControl('timeHint');
      | SampleTime=Simulink.data.evalinGlobal(bdroot,get_param(gcb,'SampleTime'));
      | SampleTime_1=str2double(get_param(gcb,'SampleTime_1'));
      | if (((SampleTime==-1) && (~contains(hintText.Prompt,'inherited'))) || ...
      |     ((SampleTime~=-1) && contains(hintText.Prompt,'inherited')) || ...
      |     ((SampleTime~=-1) && (SampleTime_1~=SampleTime)) || ...
      |     ((SampleTime_1~=-1) && contains(hintText.Prompt,'yet')))
      |   if ((SampleTime==-1) && (~contains(hintText.Prompt,'inherited')))
      |     set_param(gcb,'SampleTime_1',num2str(NaN));
      |     SampleTime_1=NaN;
      |   end
      |   if (SampleTime~=-1)
      |     set_param(gcb,'SampleTime_1',num2str(SampleTime));
      |     SampleTime_1=SampleTime;
      |   end
      |   autoCalcEn=get_param(gcb,'autoCalcEn');
      |   if strcmp(autoCalcEn,'on')
      |     p=Simulink.Mask.get(gcb);
      |     hintText=p.getDialogControl('timeHint');
      |     if SampleTime==-1
      |       SampleTime=SampleTime_1;
      |       if isnan(SampleTime)
      |         hintText.Prompt='Note: Implementation parameters cannot be calculated yet because the block''s inherited sample time is unknown. Simulink will update the sample time when you run the simulation.';
      |       else
      |         hintText.Prompt='Caution: Implementation parameters depend on inherited sample time. Make sure that the sample time of the block''s inputs corresponds to the sampling period in the target application.';
      |       end
      |     else
      |       hintText.Prompt='Caution: Implementation parameters depend on the sample time. Make sure that the simulation time step corresponds to the sampling period in the target application.';
      |     end
      |     fltUmaxDivImax_bkup=get_param(gcb,'fltUmaxDivImax');
      |     fltLambdaW_bkup=get_param(gcb,'fltLambdaW');
      |     fltLambdaFW_bkup=get_param(gcb,'fltLambdaFW');
      |     fltPropGainQ_bkup=get_param(gcb,'fltPropGainQ');
      |     fltIntegGainQ_bkup=get_param(gcb,'fltIntegGainQ');
      |     fltLowerLimitQ_bkup=get_param(gcb,'fltLowerLimitQ');
      |     fltUpperLimitQ_bkup=get_param(gcb,'fltUpperLimitQ');
      |     fltPropGainFW_bkup=get_param(gcb,'fltPropGainFW');
      |     fltIntegGainFW_bkup=get_param(gcb,'fltIntegGainFW');
      |     fltLowerLimitFW_bkup=get_param(gcb,'fltLowerLimitFW');
      |     fltUpperLimitFW_bkup=get_param(gcb,'fltUpperLimitFW');
      |     fltRampUp_bkup=get_param(gcb,'fltRampUp');
      |     fltRampDown_bkup=get_param(gcb,'fltRampDown');
      |     wf0=Simulink.data.evalinGlobal(bdroot,get_param(gcb,'wf0'));
      |     wksi=Simulink.data.evalinGlobal(bdroot,get_param(gcb,'wksi'));
      |     J=Simulink.data.evalinGlobal(bdroot,get_param(gcb,'J'));
      |     Kt=Simulink.data.evalinGlobal(bdroot,get_param(gcb,'Kt'));
      |     lambdaW=Simulink.data.evalinGlobal(bdroot,get_param(gcb,'lambdaW'));
      |     lambdaFW=Simulink.data.evalinGlobal(bdroot,get_param(gcb,'lambdaFW'));
      |     Idmax=Simulink.data.evalinGlobal(bdroot,get_param(gcb,'Idmax'));
      |     imax=Simulink.data.evalinGlobal(bdroot,get_param(gcb,'imax'));
      |     udcbus=Simulink.data.evalinGlobal(bdroot,get_param(gcb,'udcbus'));
      |     ramprpm=Simulink.data.evalinGlobal(bdroot,get_param(gcb,'ramprpm'));
      |     mechspeed=Simulink.data.evalinGlobal(bdroot,get_param(gcb,'mechspeed'));
      |     polepairs=Simulink.data.evalinGlobal(bdroot,get_param(gcb,'polepairs'));
      |     if (wf0<=0)
      |       warning('Natural frequency f0 must be positive.');
      |     end
      |     if (wksi<=0)
      |       warning('Current loop attenuation must be positive.');
      |     end
      |     if (wksi>1)
      |       warning('Current loop attenuation must not exceed 1.');
      |     end
      |     if (J<=0)
      |       warning('Moment of inertia J must be positive.');
      |     end
      |     if (Kt<=0)
      |       warning('Torque constant Kt must be positive.');
      |     end
      |     if (lambdaW<0)
      |       warning('MA filter smoothing factor must be in the range 0..1.');
      |     end
      |     if (lambdaW>1)
      |       warning('MA filter smoothing factor must be in the range 0..1.');
      |     end
      |     if (lambdaFW<0)
      |       warning('MA filter smoothing factor must be in the range 0..1.');
      |     end
      |     if (lambdaFW>1)
      |       warning('MA filter smoothing factor must be in the range 0..1.');
      |     end
      |     if (udcbus<=0)
      |       warning('DC bus voltage must be positive.');
      |     end
      |     if (imax<=0)
      |       warning('Max. phase current must be positive.');
      |     end
      |     if (mechspeed<=0)
      |       warning('Max. speed must be positive.');
      |     end
      |     if (polepairs<1)
      |       warning('Number of pole pairs must be a natural number (1, 2, 3, ...).');
      |     end
      |     if (round(polepairs)~=polepairs)
      |       warning('Number of pole pairs must be a natural number (1, 2, 3, ...).');
      |     end
      |     w0=6.283185307179586*wf0;
      |     pgain=2.0*wksi*w0*J/Kt;
      |     igain=w0*w0*J/Kt;
      |     wmax=polepairs*mechspeed*0.1047197551196598;
      |     fltPropGainQ=pgain;
      |     fltIntegGainQ=igain*SampleTime*0.5;
      |     fltLowerLimitQ=-wmax;
      |     fltUpperLimitQ=wmax;
      |     fltPropGainFW=0.9*pgain;
      |     fltIntegGainFW=fltIntegGainQ;
      |     if (Idmax<0)
      |       iratio=Idmax/imax;
      |       iratio=abs(iratio);
      |       if (abs(iratio) > 1)
      |         iratio = 0;
      |       end
      |       lowlim=acos(iratio)-1.570796326794897;
      |     else
      |       lowlim=0.0;
      |     end
      |     fltLowerLimitFW=lowlim;
      |     fltUpperLimitFW=0.0;
      |     fltLambdaW=lambdaW;
      |     fltLambdaFW=lambdaFW;
      |     rampsc=polepairs*abs(ramprpm)*0.1047197551196598;
      |     fltRampUp=rampsc;
      |     fltRampDown=rampsc;
      |     fltUmaxDivImax=0.5773502691896258*udcbus/imax;
      |     if isnan(fltUmaxDivImax)
      |       if ~strcmp(fltUmaxDivImax_bkup,'0')
      |         set_param(gcb,'fltUmaxDivImax','0');
      |       end
      |     else
      |       tmps=num2str(fltUmaxDivImax);
      |       if ~strcmp(fltUmaxDivImax_bkup,tmps)
      |         set_param(gcb,'fltUmaxDivImax',tmps);
      |       end
      |     end
      |     if isnan(fltLambdaW)
      |       if ~strcmp(fltLambdaW_bkup,'0')
      |         set_param(gcb,'fltLambdaW','0');
      |       end
      |     else
      |       tmps=num2str(fltLambdaW);
      |       if ~strcmp(fltLambdaW_bkup,tmps)
      |         set_param(gcb,'fltLambdaW',tmps);
      |       end
      |     end
      |     if isnan(fltLambdaFW)
      |       if ~strcmp(fltLambdaFW_bkup,'0')
      |         set_param(gcb,'fltLambdaFW','0');
      |       end
      |     else
      |       tmps=num2str(fltLambdaFW);
      |       if ~strcmp(fltLambdaFW_bkup,tmps)
      |         set_param(gcb,'fltLambdaFW',tmps);
      |       end
      |     end
      |     if isnan(fltPropGainQ)
      |       if ~strcmp(fltPropGainQ_bkup,'0')
      |         set_param(gcb,'fltPropGainQ','0');
      |       end
      |     else
      |       tmps=num2str(fltPropGainQ);
      |       if ~strcmp(fltPropGainQ_bkup,tmps)
      |         set_param(gcb,'fltPropGainQ',tmps);
      |       end
      |     end
      |     if isnan(fltIntegGainQ)
      |       if ~strcmp(fltIntegGainQ_bkup,'0')
      |         set_param(gcb,'fltIntegGainQ','0');
      |       end
      |     else
      |       tmps=num2str(fltIntegGainQ);
      |       if ~strcmp(fltIntegGainQ_bkup,tmps)
      |         set_param(gcb,'fltIntegGainQ',tmps);
      |       end
      |     end
      |     if isnan(fltLowerLimitQ)
      |       if ~strcmp(fltLowerLimitQ_bkup,'0')
      |         set_param(gcb,'fltLowerLimitQ','0');
      |       end
      |     else
      |       tmps=num2str(fltLowerLimitQ);
      |       if ~strcmp(fltLowerLimitQ_bkup,tmps)
      |         set_param(gcb,'fltLowerLimitQ',tmps);
      |       end
      |     end
      |     if isnan(fltUpperLimitQ)
      |       if ~strcmp(fltUpperLimitQ_bkup,'0')
      |         set_param(gcb,'fltUpperLimitQ','0');
      |       end
      |     else
      |       tmps=num2str(fltUpperLimitQ);
      |       if ~strcmp(fltUpperLimitQ_bkup,tmps)
      |         set_param(gcb,'fltUpperLimitQ',tmps);
      |       end
      |     end
      |     if isnan(fltPropGainFW)
      |       if ~strcmp(fltPropGainFW_bkup,'0')
      |         set_param(gcb,'fltPropGainFW','0');
      |       end
      |     else
      |       tmps=num2str(fltPropGainFW);
      |       if ~strcmp(fltPropGainFW_bkup,tmps)
      |         set_param(gcb,'fltPropGainFW',tmps);
      |       end
      |     end
      |     if isnan(fltIntegGainFW)
      |       if ~strcmp(fltIntegGainFW_bkup,'0')
      |         set_param(gcb,'fltIntegGainFW','0');
      |       end
      |     else
      |       tmps=num2str(fltIntegGainFW);
      |       if ~strcmp(fltIntegGainFW_bkup,tmps)
      |         set_param(gcb,'fltIntegGainFW',tmps);
      |       end
      |     end
      |     if isnan(fltLowerLimitFW)
      |       if ~strcmp(fltLowerLimitFW_bkup,'0')
      |         set_param(gcb,'fltLowerLimitFW','0');
      |       end
      |     else
      |       tmps=num2str(fltLowerLimitFW);
      |       if ~strcmp(fltLowerLimitFW_bkup,tmps)
      |         set_param(gcb,'fltLowerLimitFW',tmps);
      |       end
      |     end
      |     if isnan(fltUpperLimitFW)
      |       if ~strcmp(fltUpperLimitFW_bkup,'0')
      |         set_param(gcb,'fltUpperLimitFW','0');
      |       end
      |     else
      |       tmps=num2str(fltUpperLimitFW);
      |       if ~strcmp(fltUpperLimitFW_bkup,tmps)
      |         set_param(gcb,'fltUpperLimitFW',tmps);
      |       end
      |     end
      |     if isnan(fltRampUp)
      |       if ~strcmp(fltRampUp_bkup,'0')
      |         set_param(gcb,'fltRampUp','0');
      |       end
      |     else
      |       tmps=num2str(fltRampUp);
      |       if ~strcmp(fltRampUp_bkup,tmps)
      |         set_param(gcb,'fltRampUp',tmps);
      |       end
      |     end
      |     if isnan(fltRampDown)
      |       if ~strcmp(fltRampDown_bkup,'0')
      |         set_param(gcb,'fltRampDown','0');
      |       end
      |     else
      |       tmps=num2str(fltRampDown);
      |       if ~strcmp(fltRampDown_bkup,tmps)
      |         set_param(gcb,'fltRampDown',tmps);
      |       end
      |     end
      |   end
      | end
      mask Callback wf0:
      | autoCalcEn=get_param(gcb,'autoCalcEn');
      | if strcmp(autoCalcEn,'on')
      |   SampleTime=Simulink.data.evalinGlobal(bdroot,get_param(gcb,'SampleTime'));
      |   if (SampleTime==-1)
      |     SampleTime=str2double(get_param(gcb,'SampleTime_1'));
      |   end
      |   fltUmaxDivImax_bkup=get_param(gcb,'fltUmaxDivImax');
      |   fltLambdaW_bkup=get_param(gcb,'fltLambdaW');
      |   fltLambdaFW_bkup=get_param(gcb,'fltLambdaFW');
      |   fltPropGainQ_bkup=get_param(gcb,'fltPropGainQ');
      |   fltIntegGainQ_bkup=get_param(gcb,'fltIntegGainQ');
      |   fltLowerLimitQ_bkup=get_param(gcb,'fltLowerLimitQ');
      |   fltUpperLimitQ_bkup=get_param(gcb,'fltUpperLimitQ');
      |   fltPropGainFW_bkup=get_param(gcb,'fltPropGainFW');
      |   fltIntegGainFW_bkup=get_param(gcb,'fltIntegGainFW');
      |   fltLowerLimitFW_bkup=get_param(gcb,'fltLowerLimitFW');
      |   fltUpperLimitFW_bkup=get_param(gcb,'fltUpperLimitFW');
      |   fltRampUp_bkup=get_param(gcb,'fltRampUp');
      |   fltRampDown_bkup=get_param(gcb,'fltRampDown');
      |   wf0=Simulink.data.evalinGlobal(bdroot,get_param(gcb,'wf0'));
      |   wksi=Simulink.data.evalinGlobal(bdroot,get_param(gcb,'wksi'));
      |   J=Simulink.data.evalinGlobal(bdroot,get_param(gcb,'J'));
      |   Kt=Simulink.data.evalinGlobal(bdroot,get_param(gcb,'Kt'));
      |   lambdaW=Simulink.data.evalinGlobal(bdroot,get_param(gcb,'lambdaW'));
      |   lambdaFW=Simulink.data.evalinGlobal(bdroot,get_param(gcb,'lambdaFW'));
      |   Idmax=Simulink.data.evalinGlobal(bdroot,get_param(gcb,'Idmax'));
      |   imax=Simulink.data.evalinGlobal(bdroot,get_param(gcb,'imax'));
      |   udcbus=Simulink.data.evalinGlobal(bdroot,get_param(gcb,'udcbus'));
      |   ramprpm=Simulink.data.evalinGlobal(bdroot,get_param(gcb,'ramprpm'));
      |   mechspeed=Simulink.data.evalinGlobal(bdroot,get_param(gcb,'mechspeed'));
      |   polepairs=Simulink.data.evalinGlobal(bdroot,get_param(gcb,'polepairs'));
      |   if (wf0<=0)
      |     warning('Natural frequency f0 must be positive.');
      |   end
      |   if (wksi<=0)
      |     warning('Current loop attenuation must be positive.');
      |   end
      |   if (wksi>1)
      |     warning('Current loop attenuation must not exceed 1.');
      |   end
      |   if (J<=0)
      |     warning('Moment of inertia J must be positive.');
      |   end
      |   if (Kt<=0)
      |     warning('Torque constant Kt must be positive.');
      |   end
      |   if (lambdaW<0)
      |     warning('MA filter smoothing factor must be in the range 0..1.');
      |   end
      |   if (lambdaW>1)
      |     warning('MA filter smoothing factor must be in the range 0..1.');
      |   end
      |   if (lambdaFW<0)
      |     warning('MA filter smoothing factor must be in the range 0..1.');
      |   end
      |   if (lambdaFW>1)
      |     warning('MA filter smoothing factor must be in the range 0..1.');
      |   end
      |   if (udcbus<=0)
      |     warning('DC bus voltage must be positive.');
      |   end
      |   if (imax<=0)
      |     warning('Max. phase current must be positive.');
      |   end
      |   if (mechspeed<=0)
      |     warning('Max. speed must be positive.');
      |   end
      |   if (polepairs<1)
      |     warning('Number of pole pairs must be a natural number (1, 2, 3, ...).');
      |   end
      |   if (round(polepairs)~=polepairs)
      |     warning('Number of pole pairs must be a natural number (1, 2, 3, ...).');
      |   end
      |   w0=6.283185307179586*wf0;
      |   pgain=2.0*wksi*w0*J/Kt;
      |   igain=w0*w0*J/Kt;
      |   wmax=polepairs*mechspeed*0.1047197551196598;
      |   fltPropGainQ=pgain;
      |   fltIntegGainQ=igain*SampleTime*0.5;
      |   fltLowerLimitQ=-wmax;
      |   fltUpperLimitQ=wmax;
      |   fltPropGainFW=0.9*pgain;
      |   fltIntegGainFW=fltIntegGainQ;
      |   if (Idmax<0)
      |     iratio=Idmax/imax;
      |     iratio=abs(iratio);
      |     if (abs(iratio) > 1)
      |       iratio = 0;
      |     end
      |     lowlim=acos(iratio)-1.570796326794897;
      |   else
      |     lowlim=0.0;
      |   end
      |   fltLowerLimitFW=lowlim;
      |   fltUpperLimitFW=0.0;
      |   fltLambdaW=lambdaW;
      |   fltLambdaFW=lambdaFW;
      |   rampsc=polepairs*abs(ramprpm)*0.1047197551196598;
      |   fltRampUp=rampsc;
      |   fltRampDown=rampsc;
      |   fltUmaxDivImax=0.5773502691896258*udcbus/imax;
      |   if isnan(fltUmaxDivImax)
      |     if ~strcmp(fltUmaxDivImax_bkup,'0')
      |       set_param(gcb,'fltUmaxDivImax','0');
      |     end
      |   else
      |     tmps=num2str(fltUmaxDivImax);
      |     if ~strcmp(fltUmaxDivImax_bkup,tmps)
      |       set_param(gcb,'fltUmaxDivImax',tmps);
      |     end
      |   end
      |   if isnan(fltLambdaW)
      |     if ~strcmp(fltLambdaW_bkup,'0')
      |       set_param(gcb,'fltLambdaW','0');
      |     end
      |   else
      |     tmps=num2str(fltLambdaW);
      |     if ~strcmp(fltLambdaW_bkup,tmps)
      |       set_param(gcb,'fltLambdaW',tmps);
      |     end
      |   end
      |   if isnan(fltLambdaFW)
      |     if ~strcmp(fltLambdaFW_bkup,'0')
      |       set_param(gcb,'fltLambdaFW','0');
      |     end
      |   else
      |     tmps=num2str(fltLambdaFW);
      |     if ~strcmp(fltLambdaFW_bkup,tmps)
      |       set_param(gcb,'fltLambdaFW',tmps);
      |     end
      |   end
      |   if isnan(fltPropGainQ)
      |     if ~strcmp(fltPropGainQ_bkup,'0')
      |       set_param(gcb,'fltPropGainQ','0');
      |     end
      |   else
      |     tmps=num2str(fltPropGainQ);
      |     if ~strcmp(fltPropGainQ_bkup,tmps)
      |       set_param(gcb,'fltPropGainQ',tmps);
      |     end
      |   end
      |   if isnan(fltIntegGainQ)
      |     if ~strcmp(fltIntegGainQ_bkup,'0')
      |       set_param(gcb,'fltIntegGainQ','0');
      |     end
      |   else
      |     tmps=num2str(fltIntegGainQ);
      |     if ~strcmp(fltIntegGainQ_bkup,tmps)
      |       set_param(gcb,'fltIntegGainQ',tmps);
      |     end
      |   end
      |   if isnan(fltLowerLimitQ)
      |     if ~strcmp(fltLowerLimitQ_bkup,'0')
      |       set_param(gcb,'fltLowerLimitQ','0');
      |     end
      |   else
      |     tmps=num2str(fltLowerLimitQ);
      |     if ~strcmp(fltLowerLimitQ_bkup,tmps)
      |       set_param(gcb,'fltLowerLimitQ',tmps);
      |     end
      |   end
      |   if isnan(fltUpperLimitQ)
      |     if ~strcmp(fltUpperLimitQ_bkup,'0')
      |       set_param(gcb,'fltUpperLimitQ','0');
      |     end
      |   else
      |     tmps=num2str(fltUpperLimitQ);
      |     if ~strcmp(fltUpperLimitQ_bkup,tmps)
      |       set_param(gcb,'fltUpperLimitQ',tmps);
      |     end
      |   end
      |   if isnan(fltPropGainFW)
      |     if ~strcmp(fltPropGainFW_bkup,'0')
      |       set_param(gcb,'fltPropGainFW','0');
      |     end
      |   else
      |     tmps=num2str(fltPropGainFW);
      |     if ~strcmp(fltPropGainFW_bkup,tmps)
      |       set_param(gcb,'fltPropGainFW',tmps);
      |     end
      |   end
      |   if isnan(fltIntegGainFW)
      |     if ~strcmp(fltIntegGainFW_bkup,'0')
      |       set_param(gcb,'fltIntegGainFW','0');
      |     end
      |   else
      |     tmps=num2str(fltIntegGainFW);
      |     if ~strcmp(fltIntegGainFW_bkup,tmps)
      |       set_param(gcb,'fltIntegGainFW',tmps);
      |     end
      |   end
      |   if isnan(fltLowerLimitFW)
      |     if ~strcmp(fltLowerLimitFW_bkup,'0')
      |       set_param(gcb,'fltLowerLimitFW','0');
      |     end
      |   else
      |     tmps=num2str(fltLowerLimitFW);
      |     if ~strcmp(fltLowerLimitFW_bkup,tmps)
      |       set_param(gcb,'fltLowerLimitFW',tmps);
      |     end
      |   end
      |   if isnan(fltUpperLimitFW)
      |     if ~strcmp(fltUpperLimitFW_bkup,'0')
      |       set_param(gcb,'fltUpperLimitFW','0');
      |     end
      |   else
      |     tmps=num2str(fltUpperLimitFW);
      |     if ~strcmp(fltUpperLimitFW_bkup,tmps)
      |       set_param(gcb,'fltUpperLimitFW',tmps);
      |     end
      |   end
      |   if isnan(fltRampUp)
      |     if ~strcmp(fltRampUp_bkup,'0')
      |       set_param(gcb,'fltRampUp','0');
      |     end
      |   else
      |     tmps=num2str(fltRampUp);
      |     if ~strcmp(fltRampUp_bkup,tmps)
      |       set_param(gcb,'fltRampUp',tmps);
      |     end
      |   end
      |   if isnan(fltRampDown)
      |     if ~strcmp(fltRampDown_bkup,'0')
      |       set_param(gcb,'fltRampDown','0');
      |     end
      |   else
      |     tmps=num2str(fltRampDown);
      |     if ~strcmp(fltRampDown_bkup,tmps)
      |       set_param(gcb,'fltRampDown',tmps);
      |     end
      |   end
      | end
      mask Callback wksi:
      | autoCalcEn=get_param(gcb,'autoCalcEn');
      | if strcmp(autoCalcEn,'on')
      |   SampleTime=Simulink.data.evalinGlobal(bdroot,get_param(gcb,'SampleTime'));
      |   if (SampleTime==-1)
      |     SampleTime=str2double(get_param(gcb,'SampleTime_1'));
      |   end
      |   fltUmaxDivImax_bkup=get_param(gcb,'fltUmaxDivImax');
      |   fltLambdaW_bkup=get_param(gcb,'fltLambdaW');
      |   fltLambdaFW_bkup=get_param(gcb,'fltLambdaFW');
      |   fltPropGainQ_bkup=get_param(gcb,'fltPropGainQ');
      |   fltIntegGainQ_bkup=get_param(gcb,'fltIntegGainQ');
      |   fltLowerLimitQ_bkup=get_param(gcb,'fltLowerLimitQ');
      |   fltUpperLimitQ_bkup=get_param(gcb,'fltUpperLimitQ');
      |   fltPropGainFW_bkup=get_param(gcb,'fltPropGainFW');
      |   fltIntegGainFW_bkup=get_param(gcb,'fltIntegGainFW');
      |   fltLowerLimitFW_bkup=get_param(gcb,'fltLowerLimitFW');
      |   fltUpperLimitFW_bkup=get_param(gcb,'fltUpperLimitFW');
      |   fltRampUp_bkup=get_param(gcb,'fltRampUp');
      |   fltRampDown_bkup=get_param(gcb,'fltRampDown');
      |   wf0=Simulink.data.evalinGlobal(bdroot,get_param(gcb,'wf0'));
      |   wksi=Simulink.data.evalinGlobal(bdroot,get_param(gcb,'wksi'));
      |   J=Simulink.data.evalinGlobal(bdroot,get_param(gcb,'J'));
      |   Kt=Simulink.data.evalinGlobal(bdroot,get_param(gcb,'Kt'));
      |   lambdaW=Simulink.data.evalinGlobal(bdroot,get_param(gcb,'lambdaW'));
      |   lambdaFW=Simulink.data.evalinGlobal(bdroot,get_param(gcb,'lambdaFW'));
      |   Idmax=Simulink.data.evalinGlobal(bdroot,get_param(gcb,'Idmax'));
      |   imax=Simulink.data.evalinGlobal(bdroot,get_param(gcb,'imax'));
      |   udcbus=Simulink.data.evalinGlobal(bdroot,get_param(gcb,'udcbus'));
      |   ramprpm=Simulink.data.evalinGlobal(bdroot,get_param(gcb,'ramprpm'));
      |   mechspeed=Simulink.data.evalinGlobal(bdroot,get_param(gcb,'mechspeed'));
      |   polepairs=Simulink.data.evalinGlobal(bdroot,get_param(gcb,'polepairs'));
      |   if (wf0<=0)
      |     warning('Natural frequency f0 must be positive.');
      |   end
      |   if (wksi<=0)
      |     warning('Current loop attenuation must be positive.');
      |   end
      |   if (wksi>1)
      |     warning('Current loop attenuation must not exceed 1.');
      |   end
      |   if (J<=0)
      |     warning('Moment of inertia J must be positive.');
      |   end
      |   if (Kt<=0)
      |     warning('Torque constant Kt must be positive.');
      |   end
      |   if (lambdaW<0)
      |     warning('MA filter smoothing factor must be in the range 0..1.');
      |   end
      |   if (lambdaW>1)
      |     warning('MA filter smoothing factor must be in the range 0..1.');
      |   end
      |   if (lambdaFW<0)
      |     warning('MA filter smoothing factor must be in the range 0..1.');
      |   end
      |   if (lambdaFW>1)
      |     warning('MA filter smoothing factor must be in the range 0..1.');
      |   end
      |   if (udcbus<=0)
      |     warning('DC bus voltage must be positive.');
      |   end
      |   if (imax<=0)
      |     warning('Max. phase current must be positive.');
      |   end
      |   if (mechspeed<=0)
      |     warning('Max. speed must be positive.');
      |   end
      |   if (polepairs<1)
      |     warning('Number of pole pairs must be a natural number (1, 2, 3, ...).');
      |   end
      |   if (round(polepairs)~=polepairs)
      |     warning('Number of pole pairs must be a natural number (1, 2, 3, ...).');
      |   end
      |   w0=6.283185307179586*wf0;
      |   pgain=2.0*wksi*w0*J/Kt;
      |   igain=w0*w0*J/Kt;
      |   wmax=polepairs*mechspeed*0.1047197551196598;
      |   fltPropGainQ=pgain;
      |   fltIntegGainQ=igain*SampleTime*0.5;
      |   fltLowerLimitQ=-wmax;
      |   fltUpperLimitQ=wmax;
      |   fltPropGainFW=0.9*pgain;
      |   fltIntegGainFW=fltIntegGainQ;
      |   if (Idmax<0)
      |     iratio=Idmax/imax;
      |     iratio=abs(iratio);
      |     if (abs(iratio) > 1)
      |       iratio = 0;
      |     end
      |     lowlim=acos(iratio)-1.570796326794897;
      |   else
      |     lowlim=0.0;
      |   end
      |   fltLowerLimitFW=lowlim;
      |   fltUpperLimitFW=0.0;
      |   fltLambdaW=lambdaW;
      |   fltLambdaFW=lambdaFW;
      |   rampsc=polepairs*abs(ramprpm)*0.1047197551196598;
      |   fltRampUp=rampsc;
      |   fltRampDown=rampsc;
      |   fltUmaxDivImax=0.5773502691896258*udcbus/imax;
      |   if isnan(fltUmaxDivImax)
      |     if ~strcmp(fltUmaxDivImax_bkup,'0')
      |       set_param(gcb,'fltUmaxDivImax','0');
      |     end
      |   else
      |     tmps=num2str(fltUmaxDivImax);
      |     if ~strcmp(fltUmaxDivImax_bkup,tmps)
      |       set_param(gcb,'fltUmaxDivImax',tmps);
      |     end
      |   end
      |   if isnan(fltLambdaW)
      |     if ~strcmp(fltLambdaW_bkup,'0')
      |       set_param(gcb,'fltLambdaW','0');
      |     end
      |   else
      |     tmps=num2str(fltLambdaW);
      |     if ~strcmp(fltLambdaW_bkup,tmps)
      |       set_param(gcb,'fltLambdaW',tmps);
      |     end
      |   end
      |   if isnan(fltLambdaFW)
      |     if ~strcmp(fltLambdaFW_bkup,'0')
      |       set_param(gcb,'fltLambdaFW','0');
      |     end
      |   else
      |     tmps=num2str(fltLambdaFW);
      |     if ~strcmp(fltLambdaFW_bkup,tmps)
      |       set_param(gcb,'fltLambdaFW',tmps);
      |     end
      |   end
      |   if isnan(fltPropGainQ)
      |     if ~strcmp(fltPropGainQ_bkup,'0')
      |       set_param(gcb,'fltPropGainQ','0');
      |     end
      |   else
      |     tmps=num2str(fltPropGainQ);
      |     if ~strcmp(fltPropGainQ_bkup,tmps)
      |       set_param(gcb,'fltPropGainQ',tmps);
      |     end
      |   end
      |   if isnan(fltIntegGainQ)
      |     if ~strcmp(fltIntegGainQ_bkup,'0')
      |       set_param(gcb,'fltIntegGainQ','0');
      |     end
      |   else
      |     tmps=num2str(fltIntegGainQ);
      |     if ~strcmp(fltIntegGainQ_bkup,tmps)
      |       set_param(gcb,'fltIntegGainQ',tmps);
      |     end
      |   end
      |   if isnan(fltLowerLimitQ)
      |     if ~strcmp(fltLowerLimitQ_bkup,'0')
      |       set_param(gcb,'fltLowerLimitQ','0');
      |     end
      |   else
      |     tmps=num2str(fltLowerLimitQ);
      |     if ~strcmp(fltLowerLimitQ_bkup,tmps)
      |       set_param(gcb,'fltLowerLimitQ',tmps);
      |     end
      |   end
      |   if isnan(fltUpperLimitQ)
      |     if ~strcmp(fltUpperLimitQ_bkup,'0')
      |       set_param(gcb,'fltUpperLimitQ','0');
      |     end
      |   else
      |     tmps=num2str(fltUpperLimitQ);
      |     if ~strcmp(fltUpperLimitQ_bkup,tmps)
      |       set_param(gcb,'fltUpperLimitQ',tmps);
      |     end
      |   end
      |   if isnan(fltPropGainFW)
      |     if ~strcmp(fltPropGainFW_bkup,'0')
      |       set_param(gcb,'fltPropGainFW','0');
      |     end
      |   else
      |     tmps=num2str(fltPropGainFW);
      |     if ~strcmp(fltPropGainFW_bkup,tmps)
      |       set_param(gcb,'fltPropGainFW',tmps);
      |     end
      |   end
      |   if isnan(fltIntegGainFW)
      |     if ~strcmp(fltIntegGainFW_bkup,'0')
      |       set_param(gcb,'fltIntegGainFW','0');
      |     end
      |   else
      |     tmps=num2str(fltIntegGainFW);
      |     if ~strcmp(fltIntegGainFW_bkup,tmps)
      |       set_param(gcb,'fltIntegGainFW',tmps);
      |     end
      |   end
      |   if isnan(fltLowerLimitFW)
      |     if ~strcmp(fltLowerLimitFW_bkup,'0')
      |       set_param(gcb,'fltLowerLimitFW','0');
      |     end
      |   else
      |     tmps=num2str(fltLowerLimitFW);
      |     if ~strcmp(fltLowerLimitFW_bkup,tmps)
      |       set_param(gcb,'fltLowerLimitFW',tmps);
      |     end
      |   end
      |   if isnan(fltUpperLimitFW)
      |     if ~strcmp(fltUpperLimitFW_bkup,'0')
      |       set_param(gcb,'fltUpperLimitFW','0');
      |     end
      |   else
      |     tmps=num2str(fltUpperLimitFW);
      |     if ~strcmp(fltUpperLimitFW_bkup,tmps)
      |       set_param(gcb,'fltUpperLimitFW',tmps);
      |     end
      |   end
      |   if isnan(fltRampUp)
      |     if ~strcmp(fltRampUp_bkup,'0')
      |       set_param(gcb,'fltRampUp','0');
      |     end
      |   else
      |     tmps=num2str(fltRampUp);
      |     if ~strcmp(fltRampUp_bkup,tmps)
      |       set_param(gcb,'fltRampUp',tmps);
      |     end
      |   end
      |   if isnan(fltRampDown)
      |     if ~strcmp(fltRampDown_bkup,'0')
      |       set_param(gcb,'fltRampDown','0');
      |     end
      |   else
      |     tmps=num2str(fltRampDown);
      |     if ~strcmp(fltRampDown_bkup,tmps)
      |       set_param(gcb,'fltRampDown',tmps);
      |     end
      |   end
      | end
      mask Callback J:
      | autoCalcEn=get_param(gcb,'autoCalcEn');
      | if strcmp(autoCalcEn,'on')
      |   SampleTime=Simulink.data.evalinGlobal(bdroot,get_param(gcb,'SampleTime'));
      |   if (SampleTime==-1)
      |     SampleTime=str2double(get_param(gcb,'SampleTime_1'));
      |   end
      |   fltUmaxDivImax_bkup=get_param(gcb,'fltUmaxDivImax');
      |   fltLambdaW_bkup=get_param(gcb,'fltLambdaW');
      |   fltLambdaFW_bkup=get_param(gcb,'fltLambdaFW');
      |   fltPropGainQ_bkup=get_param(gcb,'fltPropGainQ');
      |   fltIntegGainQ_bkup=get_param(gcb,'fltIntegGainQ');
      |   fltLowerLimitQ_bkup=get_param(gcb,'fltLowerLimitQ');
      |   fltUpperLimitQ_bkup=get_param(gcb,'fltUpperLimitQ');
      |   fltPropGainFW_bkup=get_param(gcb,'fltPropGainFW');
      |   fltIntegGainFW_bkup=get_param(gcb,'fltIntegGainFW');
      |   fltLowerLimitFW_bkup=get_param(gcb,'fltLowerLimitFW');
      |   fltUpperLimitFW_bkup=get_param(gcb,'fltUpperLimitFW');
      |   fltRampUp_bkup=get_param(gcb,'fltRampUp');
      |   fltRampDown_bkup=get_param(gcb,'fltRampDown');
      |   wf0=Simulink.data.evalinGlobal(bdroot,get_param(gcb,'wf0'));
      |   wksi=Simulink.data.evalinGlobal(bdroot,get_param(gcb,'wksi'));
      |   J=Simulink.data.evalinGlobal(bdroot,get_param(gcb,'J'));
      |   Kt=Simulink.data.evalinGlobal(bdroot,get_param(gcb,'Kt'));
      |   lambdaW=Simulink.data.evalinGlobal(bdroot,get_param(gcb,'lambdaW'));
      |   lambdaFW=Simulink.data.evalinGlobal(bdroot,get_param(gcb,'lambdaFW'));
      |   Idmax=Simulink.data.evalinGlobal(bdroot,get_param(gcb,'Idmax'));
      |   imax=Simulink.data.evalinGlobal(bdroot,get_param(gcb,'imax'));
      |   udcbus=Simulink.data.evalinGlobal(bdroot,get_param(gcb,'udcbus'));
      |   ramprpm=Simulink.data.evalinGlobal(bdroot,get_param(gcb,'ramprpm'));
      |   mechspeed=Simulink.data.evalinGlobal(bdroot,get_param(gcb,'mechspeed'));
      |   polepairs=Simulink.data.evalinGlobal(bdroot,get_param(gcb,'polepairs'));
      |   if (wf0<=0)
      |     warning('Natural frequency f0 must be positive.');
      |   end
      |   if (wksi<=0)
      |     warning('Current loop attenuation must be positive.');
      |   end
      |   if (wksi>1)
      |     warning('Current loop attenuation must not exceed 1.');
      |   end
      |   if (J<=0)
      |     warning('Moment of inertia J must be positive.');
      |   end
      |   if (Kt<=0)
      |     warning('Torque constant Kt must be positive.');
      |   end
      |   if (lambdaW<0)
      |     warning('MA filter smoothing factor must be in the range 0..1.');
      |   end
      |   if (lambdaW>1)
      |     warning('MA filter smoothing factor must be in the range 0..1.');
      |   end
      |   if (lambdaFW<0)
      |     warning('MA filter smoothing factor must be in the range 0..1.');
      |   end
      |   if (lambdaFW>1)
      |     warning('MA filter smoothing factor must be in the range 0..1.');
      |   end
      |   if (udcbus<=0)
      |     warning('DC bus voltage must be positive.');
      |   end
      |   if (imax<=0)
      |     warning('Max. phase current must be positive.');
      |   end
      |   if (mechspeed<=0)
      |     warning('Max. speed must be positive.');
      |   end
      |   if (polepairs<1)
      |     warning('Number of pole pairs must be a natural number (1, 2, 3, ...).');
      |   end
      |   if (round(polepairs)~=polepairs)
      |     warning('Number of pole pairs must be a natural number (1, 2, 3, ...).');
      |   end
      |   w0=6.283185307179586*wf0;
      |   pgain=2.0*wksi*w0*J/Kt;
      |   igain=w0*w0*J/Kt;
      |   wmax=polepairs*mechspeed*0.1047197551196598;
      |   fltPropGainQ=pgain;
      |   fltIntegGainQ=igain*SampleTime*0.5;
      |   fltLowerLimitQ=-wmax;
      |   fltUpperLimitQ=wmax;
      |   fltPropGainFW=0.9*pgain;
      |   fltIntegGainFW=fltIntegGainQ;
      |   if (Idmax<0)
      |     iratio=Idmax/imax;
      |     iratio=abs(iratio);
      |     if (abs(iratio) > 1)
      |       iratio = 0;
      |     end
      |     lowlim=acos(iratio)-1.570796326794897;
      |   else
      |     lowlim=0.0;
      |   end
      |   fltLowerLimitFW=lowlim;
      |   fltUpperLimitFW=0.0;
      |   fltLambdaW=lambdaW;
      |   fltLambdaFW=lambdaFW;
      |   rampsc=polepairs*abs(ramprpm)*0.1047197551196598;
      |   fltRampUp=rampsc;
      |   fltRampDown=rampsc;
      |   fltUmaxDivImax=0.5773502691896258*udcbus/imax;
      |   if isnan(fltUmaxDivImax)
      |     if ~strcmp(fltUmaxDivImax_bkup,'0')
      |       set_param(gcb,'fltUmaxDivImax','0');
      |     end
      |   else
      |     tmps=num2str(fltUmaxDivImax);
      |     if ~strcmp(fltUmaxDivImax_bkup,tmps)
      |       set_param(gcb,'fltUmaxDivImax',tmps);
      |     end
      |   end
      |   if isnan(fltLambdaW)
      |     if ~strcmp(fltLambdaW_bkup,'0')
      |       set_param(gcb,'fltLambdaW','0');
      |     end
      |   else
      |     tmps=num2str(fltLambdaW);
      |     if ~strcmp(fltLambdaW_bkup,tmps)
      |       set_param(gcb,'fltLambdaW',tmps);
      |     end
      |   end
      |   if isnan(fltLambdaFW)
      |     if ~strcmp(fltLambdaFW_bkup,'0')
      |       set_param(gcb,'fltLambdaFW','0');
      |     end
      |   else
      |     tmps=num2str(fltLambdaFW);
      |     if ~strcmp(fltLambdaFW_bkup,tmps)
      |       set_param(gcb,'fltLambdaFW',tmps);
      |     end
      |   end
      |   if isnan(fltPropGainQ)
      |     if ~strcmp(fltPropGainQ_bkup,'0')
      |       set_param(gcb,'fltPropGainQ','0');
      |     end
      |   else
      |     tmps=num2str(fltPropGainQ);
      |     if ~strcmp(fltPropGainQ_bkup,tmps)
      |       set_param(gcb,'fltPropGainQ',tmps);
      |     end
      |   end
      |   if isnan(fltIntegGainQ)
      |     if ~strcmp(fltIntegGainQ_bkup,'0')
      |       set_param(gcb,'fltIntegGainQ','0');
      |     end
      |   else
      |     tmps=num2str(fltIntegGainQ);
      |     if ~strcmp(fltIntegGainQ_bkup,tmps)
      |       set_param(gcb,'fltIntegGainQ',tmps);
      |     end
      |   end
      |   if isnan(fltLowerLimitQ)
      |     if ~strcmp(fltLowerLimitQ_bkup,'0')
      |       set_param(gcb,'fltLowerLimitQ','0');
      |     end
      |   else
      |     tmps=num2str(fltLowerLimitQ);
      |     if ~strcmp(fltLowerLimitQ_bkup,tmps)
      |       set_param(gcb,'fltLowerLimitQ',tmps);
      |     end
      |   end
      |   if isnan(fltUpperLimitQ)
      |     if ~strcmp(fltUpperLimitQ_bkup,'0')
      |       set_param(gcb,'fltUpperLimitQ','0');
      |     end
      |   else
      |     tmps=num2str(fltUpperLimitQ);
      |     if ~strcmp(fltUpperLimitQ_bkup,tmps)
      |       set_param(gcb,'fltUpperLimitQ',tmps);
      |     end
      |   end
      |   if isnan(fltPropGainFW)
      |     if ~strcmp(fltPropGainFW_bkup,'0')
      |       set_param(gcb,'fltPropGainFW','0');
      |     end
      |   else
      |     tmps=num2str(fltPropGainFW);
      |     if ~strcmp(fltPropGainFW_bkup,tmps)
      |       set_param(gcb,'fltPropGainFW',tmps);
      |     end
      |   end
      |   if isnan(fltIntegGainFW)
      |     if ~strcmp(fltIntegGainFW_bkup,'0')
      |       set_param(gcb,'fltIntegGainFW','0');
      |     end
      |   else
      |     tmps=num2str(fltIntegGainFW);
      |     if ~strcmp(fltIntegGainFW_bkup,tmps)
      |       set_param(gcb,'fltIntegGainFW',tmps);
      |     end
      |   end
      |   if isnan(fltLowerLimitFW)
      |     if ~strcmp(fltLowerLimitFW_bkup,'0')
      |       set_param(gcb,'fltLowerLimitFW','0');
      |     end
      |   else
      |     tmps=num2str(fltLowerLimitFW);
      |     if ~strcmp(fltLowerLimitFW_bkup,tmps)
      |       set_param(gcb,'fltLowerLimitFW',tmps);
      |     end
      |   end
      |   if isnan(fltUpperLimitFW)
      |     if ~strcmp(fltUpperLimitFW_bkup,'0')
      |       set_param(gcb,'fltUpperLimitFW','0');
      |     end
      |   else
      |     tmps=num2str(fltUpperLimitFW);
      |     if ~strcmp(fltUpperLimitFW_bkup,tmps)
      |       set_param(gcb,'fltUpperLimitFW',tmps);
      |     end
      |   end
      |   if isnan(fltRampUp)
      |     if ~strcmp(fltRampUp_bkup,'0')
      |       set_param(gcb,'fltRampUp','0');
      |     end
      |   else
      |     tmps=num2str(fltRampUp);
      |     if ~strcmp(fltRampUp_bkup,tmps)
      |       set_param(gcb,'fltRampUp',tmps);
      |     end
      |   end
      |   if isnan(fltRampDown)
      |     if ~strcmp(fltRampDown_bkup,'0')
      |       set_param(gcb,'fltRampDown','0');
      |     end
      |   else
      |     tmps=num2str(fltRampDown);
      |     if ~strcmp(fltRampDown_bkup,tmps)
      |       set_param(gcb,'fltRampDown',tmps);
      |     end
      |   end
      | end
      mask Callback Kt:
      | autoCalcEn=get_param(gcb,'autoCalcEn');
      | if strcmp(autoCalcEn,'on')
      |   SampleTime=Simulink.data.evalinGlobal(bdroot,get_param(gcb,'SampleTime'));
      |   if (SampleTime==-1)
      |     SampleTime=str2double(get_param(gcb,'SampleTime_1'));
      |   end
      |   fltUmaxDivImax_bkup=get_param(gcb,'fltUmaxDivImax');
      |   fltLambdaW_bkup=get_param(gcb,'fltLambdaW');
      |   fltLambdaFW_bkup=get_param(gcb,'fltLambdaFW');
      |   fltPropGainQ_bkup=get_param(gcb,'fltPropGainQ');
      |   fltIntegGainQ_bkup=get_param(gcb,'fltIntegGainQ');
      |   fltLowerLimitQ_bkup=get_param(gcb,'fltLowerLimitQ');
      |   fltUpperLimitQ_bkup=get_param(gcb,'fltUpperLimitQ');
      |   fltPropGainFW_bkup=get_param(gcb,'fltPropGainFW');
      |   fltIntegGainFW_bkup=get_param(gcb,'fltIntegGainFW');
      |   fltLowerLimitFW_bkup=get_param(gcb,'fltLowerLimitFW');
      |   fltUpperLimitFW_bkup=get_param(gcb,'fltUpperLimitFW');
      |   fltRampUp_bkup=get_param(gcb,'fltRampUp');
      |   fltRampDown_bkup=get_param(gcb,'fltRampDown');
      |   wf0=Simulink.data.evalinGlobal(bdroot,get_param(gcb,'wf0'));
      |   wksi=Simulink.data.evalinGlobal(bdroot,get_param(gcb,'wksi'));
      |   J=Simulink.data.evalinGlobal(bdroot,get_param(gcb,'J'));
      |   Kt=Simulink.data.evalinGlobal(bdroot,get_param(gcb,'Kt'));
      |   lambdaW=Simulink.data.evalinGlobal(bdroot,get_param(gcb,'lambdaW'));
      |   lambdaFW=Simulink.data.evalinGlobal(bdroot,get_param(gcb,'lambdaFW'));
      |   Idmax=Simulink.data.evalinGlobal(bdroot,get_param(gcb,'Idmax'));
      |   imax=Simulink.data.evalinGlobal(bdroot,get_param(gcb,'imax'));
      |   udcbus=Simulink.data.evalinGlobal(bdroot,get_param(gcb,'udcbus'));
      |   ramprpm=Simulink.data.evalinGlobal(bdroot,get_param(gcb,'ramprpm'));
      |   mechspeed=Simulink.data.evalinGlobal(bdroot,get_param(gcb,'mechspeed'));
      |   polepairs=Simulink.data.evalinGlobal(bdroot,get_param(gcb,'polepairs'));
      |   if (wf0<=0)
      |     warning('Natural frequency f0 must be positive.');
      |   end
      |   if (wksi<=0)
      |     warning('Current loop attenuation must be positive.');
      |   end
      |   if (wksi>1)
      |     warning('Current loop attenuation must not exceed 1.');
      |   end
      |   if (J<=0)
      |     warning('Moment of inertia J must be positive.');
      |   end
      |   if (Kt<=0)
      |     warning('Torque constant Kt must be positive.');
      |   end
      |   if (lambdaW<0)
      |     warning('MA filter smoothing factor must be in the range 0..1.');
      |   end
      |   if (lambdaW>1)
      |     warning('MA filter smoothing factor must be in the range 0..1.');
      |   end
      |   if (lambdaFW<0)
      |     warning('MA filter smoothing factor must be in the range 0..1.');
      |   end
      |   if (lambdaFW>1)
      |     warning('MA filter smoothing factor must be in the range 0..1.');
      |   end
      |   if (udcbus<=0)
      |     warning('DC bus voltage must be positive.');
      |   end
      |   if (imax<=0)
      |     warning('Max. phase current must be positive.');
      |   end
      |   if (mechspeed<=0)
      |     warning('Max. speed must be positive.');
      |   end
      |   if (polepairs<1)
      |     warning('Number of pole pairs must be a natural number (1, 2, 3, ...).');
      |   end
      |   if (round(polepairs)~=polepairs)
      |     warning('Number of pole pairs must be a natural number (1, 2, 3, ...).');
      |   end
      |   w0=6.283185307179586*wf0;
      |   pgain=2.0*wksi*w0*J/Kt;
      |   igain=w0*w0*J/Kt;
      |   wmax=polepairs*mechspeed*0.1047197551196598;
      |   fltPropGainQ=pgain;
      |   fltIntegGainQ=igain*SampleTime*0.5;
      |   fltLowerLimitQ=-wmax;
      |   fltUpperLimitQ=wmax;
      |   fltPropGainFW=0.9*pgain;
      |   fltIntegGainFW=fltIntegGainQ;
      |   if (Idmax<0)
      |     iratio=Idmax/imax;
      |     iratio=abs(iratio);
      |     if (abs(iratio) > 1)
      |       iratio = 0;
      |     end
      |     lowlim=acos(iratio)-1.570796326794897;
      |   else
      |     lowlim=0.0;
      |   end
      |   fltLowerLimitFW=lowlim;
      |   fltUpperLimitFW=0.0;
      |   fltLambdaW=lambdaW;
      |   fltLambdaFW=lambdaFW;
      |   rampsc=polepairs*abs(ramprpm)*0.1047197551196598;
      |   fltRampUp=rampsc;
      |   fltRampDown=rampsc;
      |   fltUmaxDivImax=0.5773502691896258*udcbus/imax;
      |   if isnan(fltUmaxDivImax)
      |     if ~strcmp(fltUmaxDivImax_bkup,'0')
      |       set_param(gcb,'fltUmaxDivImax','0');
      |     end
      |   else
      |     tmps=num2str(fltUmaxDivImax);
      |     if ~strcmp(fltUmaxDivImax_bkup,tmps)
      |       set_param(gcb,'fltUmaxDivImax',tmps);
      |     end
      |   end
      |   if isnan(fltLambdaW)
      |     if ~strcmp(fltLambdaW_bkup,'0')
      |       set_param(gcb,'fltLambdaW','0');
      |     end
      |   else
      |     tmps=num2str(fltLambdaW);
      |     if ~strcmp(fltLambdaW_bkup,tmps)
      |       set_param(gcb,'fltLambdaW',tmps);
      |     end
      |   end
      |   if isnan(fltLambdaFW)
      |     if ~strcmp(fltLambdaFW_bkup,'0')
      |       set_param(gcb,'fltLambdaFW','0');
      |     end
      |   else
      |     tmps=num2str(fltLambdaFW);
      |     if ~strcmp(fltLambdaFW_bkup,tmps)
      |       set_param(gcb,'fltLambdaFW',tmps);
      |     end
      |   end
      |   if isnan(fltPropGainQ)
      |     if ~strcmp(fltPropGainQ_bkup,'0')
      |       set_param(gcb,'fltPropGainQ','0');
      |     end
      |   else
      |     tmps=num2str(fltPropGainQ);
      |     if ~strcmp(fltPropGainQ_bkup,tmps)
      |       set_param(gcb,'fltPropGainQ',tmps);
      |     end
      |   end
      |   if isnan(fltIntegGainQ)
      |     if ~strcmp(fltIntegGainQ_bkup,'0')
      |       set_param(gcb,'fltIntegGainQ','0');
      |     end
      |   else
      |     tmps=num2str(fltIntegGainQ);
      |     if ~strcmp(fltIntegGainQ_bkup,tmps)
      |       set_param(gcb,'fltIntegGainQ',tmps);
      |     end
      |   end
      |   if isnan(fltLowerLimitQ)
      |     if ~strcmp(fltLowerLimitQ_bkup,'0')
      |       set_param(gcb,'fltLowerLimitQ','0');
      |     end
      |   else
      |     tmps=num2str(fltLowerLimitQ);
      |     if ~strcmp(fltLowerLimitQ_bkup,tmps)
      |       set_param(gcb,'fltLowerLimitQ',tmps);
      |     end
      |   end
      |   if isnan(fltUpperLimitQ)
      |     if ~strcmp(fltUpperLimitQ_bkup,'0')
      |       set_param(gcb,'fltUpperLimitQ','0');
      |     end
      |   else
      |     tmps=num2str(fltUpperLimitQ);
      |     if ~strcmp(fltUpperLimitQ_bkup,tmps)
      |       set_param(gcb,'fltUpperLimitQ',tmps);
      |     end
      |   end
      |   if isnan(fltPropGainFW)
      |     if ~strcmp(fltPropGainFW_bkup,'0')
      |       set_param(gcb,'fltPropGainFW','0');
      |     end
      |   else
      |     tmps=num2str(fltPropGainFW);
      |     if ~strcmp(fltPropGainFW_bkup,tmps)
      |       set_param(gcb,'fltPropGainFW',tmps);
      |     end
      |   end
      |   if isnan(fltIntegGainFW)
      |     if ~strcmp(fltIntegGainFW_bkup,'0')
      |       set_param(gcb,'fltIntegGainFW','0');
      |     end
      |   else
      |     tmps=num2str(fltIntegGainFW);
      |     if ~strcmp(fltIntegGainFW_bkup,tmps)
      |       set_param(gcb,'fltIntegGainFW',tmps);
      |     end
      |   end
      |   if isnan(fltLowerLimitFW)
      |     if ~strcmp(fltLowerLimitFW_bkup,'0')
      |       set_param(gcb,'fltLowerLimitFW','0');
      |     end
      |   else
      |     tmps=num2str(fltLowerLimitFW);
      |     if ~strcmp(fltLowerLimitFW_bkup,tmps)
      |       set_param(gcb,'fltLowerLimitFW',tmps);
      |     end
      |   end
      |   if isnan(fltUpperLimitFW)
      |     if ~strcmp(fltUpperLimitFW_bkup,'0')
      |       set_param(gcb,'fltUpperLimitFW','0');
      |     end
      |   else
      |     tmps=num2str(fltUpperLimitFW);
      |     if ~strcmp(fltUpperLimitFW_bkup,tmps)
      |       set_param(gcb,'fltUpperLimitFW',tmps);
      |     end
      |   end
      |   if isnan(fltRampUp)
      |     if ~strcmp(fltRampUp_bkup,'0')
      |       set_param(gcb,'fltRampUp','0');
      |     end
      |   else
      |     tmps=num2str(fltRampUp);
      |     if ~strcmp(fltRampUp_bkup,tmps)
      |       set_param(gcb,'fltRampUp',tmps);
      |     end
      |   end
      |   if isnan(fltRampDown)
      |     if ~strcmp(fltRampDown_bkup,'0')
      |       set_param(gcb,'fltRampDown','0');
      |     end
      |   else
      |     tmps=num2str(fltRampDown);
      |     if ~strcmp(fltRampDown_bkup,tmps)
      |       set_param(gcb,'fltRampDown',tmps);
      |     end
      |   end
      | end
      mask Callback lambdaW:
      | autoCalcEn=get_param(gcb,'autoCalcEn');
      | if strcmp(autoCalcEn,'on')
      |   SampleTime=Simulink.data.evalinGlobal(bdroot,get_param(gcb,'SampleTime'));
      |   if (SampleTime==-1)
      |     SampleTime=str2double(get_param(gcb,'SampleTime_1'));
      |   end
      |   fltUmaxDivImax_bkup=get_param(gcb,'fltUmaxDivImax');
      |   fltLambdaW_bkup=get_param(gcb,'fltLambdaW');
      |   fltLambdaFW_bkup=get_param(gcb,'fltLambdaFW');
      |   fltPropGainQ_bkup=get_param(gcb,'fltPropGainQ');
      |   fltIntegGainQ_bkup=get_param(gcb,'fltIntegGainQ');
      |   fltLowerLimitQ_bkup=get_param(gcb,'fltLowerLimitQ');
      |   fltUpperLimitQ_bkup=get_param(gcb,'fltUpperLimitQ');
      |   fltPropGainFW_bkup=get_param(gcb,'fltPropGainFW');
      |   fltIntegGainFW_bkup=get_param(gcb,'fltIntegGainFW');
      |   fltLowerLimitFW_bkup=get_param(gcb,'fltLowerLimitFW');
      |   fltUpperLimitFW_bkup=get_param(gcb,'fltUpperLimitFW');
      |   fltRampUp_bkup=get_param(gcb,'fltRampUp');
      |   fltRampDown_bkup=get_param(gcb,'fltRampDown');
      |   wf0=Simulink.data.evalinGlobal(bdroot,get_param(gcb,'wf0'));
      |   wksi=Simulink.data.evalinGlobal(bdroot,get_param(gcb,'wksi'));
      |   J=Simulink.data.evalinGlobal(bdroot,get_param(gcb,'J'));
      |   Kt=Simulink.data.evalinGlobal(bdroot,get_param(gcb,'Kt'));
      |   lambdaW=Simulink.data.evalinGlobal(bdroot,get_param(gcb,'lambdaW'));
      |   lambdaFW=Simulink.data.evalinGlobal(bdroot,get_param(gcb,'lambdaFW'));
      |   Idmax=Simulink.data.evalinGlobal(bdroot,get_param(gcb,'Idmax'));
      |   imax=Simulink.data.evalinGlobal(bdroot,get_param(gcb,'imax'));
      |   udcbus=Simulink.data.evalinGlobal(bdroot,get_param(gcb,'udcbus'));
      |   ramprpm=Simulink.data.evalinGlobal(bdroot,get_param(gcb,'ramprpm'));
      |   mechspeed=Simulink.data.evalinGlobal(bdroot,get_param(gcb,'mechspeed'));
      |   polepairs=Simulink.data.evalinGlobal(bdroot,get_param(gcb,'polepairs'));
      |   if (wf0<=0)
      |     warning('Natural frequency f0 must be positive.');
      |   end
      |   if (wksi<=0)
      |     warning('Current loop attenuation must be positive.');
      |   end
      |   if (wksi>1)
      |     warning('Current loop attenuation must not exceed 1.');
      |   end
      |   if (J<=0)
      |     warning('Moment of inertia J must be positive.');
      |   end
      |   if (Kt<=0)
      |     warning('Torque constant Kt must be positive.');
      |   end
      |   if (lambdaW<0)
      |     warning('MA filter smoothing factor must be in the range 0..1.');
      |   end
      |   if (lambdaW>1)
      |     warning('MA filter smoothing factor must be in the range 0..1.');
      |   end
      |   if (lambdaFW<0)
      |     warning('MA filter smoothing factor must be in the range 0..1.');
      |   end
      |   if (lambdaFW>1)
      |     warning('MA filter smoothing factor must be in the range 0..1.');
      |   end
      |   if (udcbus<=0)
      |     warning('DC bus voltage must be positive.');
      |   end
      |   if (imax<=0)
      |     warning('Max. phase current must be positive.');
      |   end
      |   if (mechspeed<=0)
      |     warning('Max. speed must be positive.');
      |   end
      |   if (polepairs<1)
      |     warning('Number of pole pairs must be a natural number (1, 2, 3, ...).');
      |   end
      |   if (round(polepairs)~=polepairs)
      |     warning('Number of pole pairs must be a natural number (1, 2, 3, ...).');
      |   end
      |   w0=6.283185307179586*wf0;
      |   pgain=2.0*wksi*w0*J/Kt;
      |   igain=w0*w0*J/Kt;
      |   wmax=polepairs*mechspeed*0.1047197551196598;
      |   fltPropGainQ=pgain;
      |   fltIntegGainQ=igain*SampleTime*0.5;
      |   fltLowerLimitQ=-wmax;
      |   fltUpperLimitQ=wmax;
      |   fltPropGainFW=0.9*pgain;
      |   fltIntegGainFW=fltIntegGainQ;
      |   if (Idmax<0)
      |     iratio=Idmax/imax;
      |     iratio=abs(iratio);
      |     if (abs(iratio) > 1)
      |       iratio = 0;
      |     end
      |     lowlim=acos(iratio)-1.570796326794897;
      |   else
      |     lowlim=0.0;
      |   end
      |   fltLowerLimitFW=lowlim;
      |   fltUpperLimitFW=0.0;
      |   fltLambdaW=lambdaW;
      |   fltLambdaFW=lambdaFW;
      |   rampsc=polepairs*abs(ramprpm)*0.1047197551196598;
      |   fltRampUp=rampsc;
      |   fltRampDown=rampsc;
      |   fltUmaxDivImax=0.5773502691896258*udcbus/imax;
      |   if isnan(fltUmaxDivImax)
      |     if ~strcmp(fltUmaxDivImax_bkup,'0')
      |       set_param(gcb,'fltUmaxDivImax','0');
      |     end
      |   else
      |     tmps=num2str(fltUmaxDivImax);
      |     if ~strcmp(fltUmaxDivImax_bkup,tmps)
      |       set_param(gcb,'fltUmaxDivImax',tmps);
      |     end
      |   end
      |   if isnan(fltLambdaW)
      |     if ~strcmp(fltLambdaW_bkup,'0')
      |       set_param(gcb,'fltLambdaW','0');
      |     end
      |   else
      |     tmps=num2str(fltLambdaW);
      |     if ~strcmp(fltLambdaW_bkup,tmps)
      |       set_param(gcb,'fltLambdaW',tmps);
      |     end
      |   end
      |   if isnan(fltLambdaFW)
      |     if ~strcmp(fltLambdaFW_bkup,'0')
      |       set_param(gcb,'fltLambdaFW','0');
      |     end
      |   else
      |     tmps=num2str(fltLambdaFW);
      |     if ~strcmp(fltLambdaFW_bkup,tmps)
      |       set_param(gcb,'fltLambdaFW',tmps);
      |     end
      |   end
      |   if isnan(fltPropGainQ)
      |     if ~strcmp(fltPropGainQ_bkup,'0')
      |       set_param(gcb,'fltPropGainQ','0');
      |     end
      |   else
      |     tmps=num2str(fltPropGainQ);
      |     if ~strcmp(fltPropGainQ_bkup,tmps)
      |       set_param(gcb,'fltPropGainQ',tmps);
      |     end
      |   end
      |   if isnan(fltIntegGainQ)
      |     if ~strcmp(fltIntegGainQ_bkup,'0')
      |       set_param(gcb,'fltIntegGainQ','0');
      |     end
      |   else
      |     tmps=num2str(fltIntegGainQ);
      |     if ~strcmp(fltIntegGainQ_bkup,tmps)
      |       set_param(gcb,'fltIntegGainQ',tmps);
      |     end
      |   end
      |   if isnan(fltLowerLimitQ)
      |     if ~strcmp(fltLowerLimitQ_bkup,'0')
      |       set_param(gcb,'fltLowerLimitQ','0');
      |     end
      |   else
      |     tmps=num2str(fltLowerLimitQ);
      |     if ~strcmp(fltLowerLimitQ_bkup,tmps)
      |       set_param(gcb,'fltLowerLimitQ',tmps);
      |     end
      |   end
      |   if isnan(fltUpperLimitQ)
      |     if ~strcmp(fltUpperLimitQ_bkup,'0')
      |       set_param(gcb,'fltUpperLimitQ','0');
      |     end
      |   else
      |     tmps=num2str(fltUpperLimitQ);
      |     if ~strcmp(fltUpperLimitQ_bkup,tmps)
      |       set_param(gcb,'fltUpperLimitQ',tmps);
      |     end
      |   end
      |   if isnan(fltPropGainFW)
      |     if ~strcmp(fltPropGainFW_bkup,'0')
      |       set_param(gcb,'fltPropGainFW','0');
      |     end
      |   else
      |     tmps=num2str(fltPropGainFW);
      |     if ~strcmp(fltPropGainFW_bkup,tmps)
      |       set_param(gcb,'fltPropGainFW',tmps);
      |     end
      |   end
      |   if isnan(fltIntegGainFW)
      |     if ~strcmp(fltIntegGainFW_bkup,'0')
      |       set_param(gcb,'fltIntegGainFW','0');
      |     end
      |   else
      |     tmps=num2str(fltIntegGainFW);
      |     if ~strcmp(fltIntegGainFW_bkup,tmps)
      |       set_param(gcb,'fltIntegGainFW',tmps);
      |     end
      |   end
      |   if isnan(fltLowerLimitFW)
      |     if ~strcmp(fltLowerLimitFW_bkup,'0')
      |       set_param(gcb,'fltLowerLimitFW','0');
      |     end
      |   else
      |     tmps=num2str(fltLowerLimitFW);
      |     if ~strcmp(fltLowerLimitFW_bkup,tmps)
      |       set_param(gcb,'fltLowerLimitFW',tmps);
      |     end
      |   end
      |   if isnan(fltUpperLimitFW)
      |     if ~strcmp(fltUpperLimitFW_bkup,'0')
      |       set_param(gcb,'fltUpperLimitFW','0');
      |     end
      |   else
      |     tmps=num2str(fltUpperLimitFW);
      |     if ~strcmp(fltUpperLimitFW_bkup,tmps)
      |       set_param(gcb,'fltUpperLimitFW',tmps);
      |     end
      |   end
      |   if isnan(fltRampUp)
      |     if ~strcmp(fltRampUp_bkup,'0')
      |       set_param(gcb,'fltRampUp','0');
      |     end
      |   else
      |     tmps=num2str(fltRampUp);
      |     if ~strcmp(fltRampUp_bkup,tmps)
      |       set_param(gcb,'fltRampUp',tmps);
      |     end
      |   end
      |   if isnan(fltRampDown)
      |     if ~strcmp(fltRampDown_bkup,'0')
      |       set_param(gcb,'fltRampDown','0');
      |     end
      |   else
      |     tmps=num2str(fltRampDown);
      |     if ~strcmp(fltRampDown_bkup,tmps)
      |       set_param(gcb,'fltRampDown',tmps);
      |     end
      |   end
      | end
      mask Callback lambdaFW:
      | autoCalcEn=get_param(gcb,'autoCalcEn');
      | if strcmp(autoCalcEn,'on')
      |   SampleTime=Simulink.data.evalinGlobal(bdroot,get_param(gcb,'SampleTime'));
      |   if (SampleTime==-1)
      |     SampleTime=str2double(get_param(gcb,'SampleTime_1'));
      |   end
      |   fltUmaxDivImax_bkup=get_param(gcb,'fltUmaxDivImax');
      |   fltLambdaW_bkup=get_param(gcb,'fltLambdaW');
      |   fltLambdaFW_bkup=get_param(gcb,'fltLambdaFW');
      |   fltPropGainQ_bkup=get_param(gcb,'fltPropGainQ');
      |   fltIntegGainQ_bkup=get_param(gcb,'fltIntegGainQ');
      |   fltLowerLimitQ_bkup=get_param(gcb,'fltLowerLimitQ');
      |   fltUpperLimitQ_bkup=get_param(gcb,'fltUpperLimitQ');
      |   fltPropGainFW_bkup=get_param(gcb,'fltPropGainFW');
      |   fltIntegGainFW_bkup=get_param(gcb,'fltIntegGainFW');
      |   fltLowerLimitFW_bkup=get_param(gcb,'fltLowerLimitFW');
      |   fltUpperLimitFW_bkup=get_param(gcb,'fltUpperLimitFW');
      |   fltRampUp_bkup=get_param(gcb,'fltRampUp');
      |   fltRampDown_bkup=get_param(gcb,'fltRampDown');
      |   wf0=Simulink.data.evalinGlobal(bdroot,get_param(gcb,'wf0'));
      |   wksi=Simulink.data.evalinGlobal(bdroot,get_param(gcb,'wksi'));
      |   J=Simulink.data.evalinGlobal(bdroot,get_param(gcb,'J'));
      |   Kt=Simulink.data.evalinGlobal(bdroot,get_param(gcb,'Kt'));
      |   lambdaW=Simulink.data.evalinGlobal(bdroot,get_param(gcb,'lambdaW'));
      |   lambdaFW=Simulink.data.evalinGlobal(bdroot,get_param(gcb,'lambdaFW'));
      |   Idmax=Simulink.data.evalinGlobal(bdroot,get_param(gcb,'Idmax'));
      |   imax=Simulink.data.evalinGlobal(bdroot,get_param(gcb,'imax'));
      |   udcbus=Simulink.data.evalinGlobal(bdroot,get_param(gcb,'udcbus'));
      |   ramprpm=Simulink.data.evalinGlobal(bdroot,get_param(gcb,'ramprpm'));
      |   mechspeed=Simulink.data.evalinGlobal(bdroot,get_param(gcb,'mechspeed'));
      |   polepairs=Simulink.data.evalinGlobal(bdroot,get_param(gcb,'polepairs'));
      |   if (wf0<=0)
      |     warning('Natural frequency f0 must be positive.');
      |   end
      |   if (wksi<=0)
      |     warning('Current loop attenuation must be positive.');
      |   end
      |   if (wksi>1)
      |     warning('Current loop attenuation must not exceed 1.');
      |   end
      |   if (J<=0)
      |     warning('Moment of inertia J must be positive.');
      |   end
      |   if (Kt<=0)
      |     warning('Torque constant Kt must be positive.');
      |   end
      |   if (lambdaW<0)
      |     warning('MA filter smoothing factor must be in the range 0..1.');
      |   end
      |   if (lambdaW>1)
      |     warning('MA filter smoothing factor must be in the range 0..1.');
      |   end
      |   if (lambdaFW<0)
      |     warning('MA filter smoothing factor must be in the range 0..1.');
      |   end
      |   if (lambdaFW>1)
      |     warning('MA filter smoothing factor must be in the range 0..1.');
      |   end
      |   if (udcbus<=0)
      |     warning('DC bus voltage must be positive.');
      |   end
      |   if (imax<=0)
      |     warning('Max. phase current must be positive.');
      |   end
      |   if (mechspeed<=0)
      |     warning('Max. speed must be positive.');
      |   end
      |   if (polepairs<1)
      |     warning('Number of pole pairs must be a natural number (1, 2, 3, ...).');
      |   end
      |   if (round(polepairs)~=polepairs)
      |     warning('Number of pole pairs must be a natural number (1, 2, 3, ...).');
      |   end
      |   w0=6.283185307179586*wf0;
      |   pgain=2.0*wksi*w0*J/Kt;
      |   igain=w0*w0*J/Kt;
      |   wmax=polepairs*mechspeed*0.1047197551196598;
      |   fltPropGainQ=pgain;
      |   fltIntegGainQ=igain*SampleTime*0.5;
      |   fltLowerLimitQ=-wmax;
      |   fltUpperLimitQ=wmax;
      |   fltPropGainFW=0.9*pgain;
      |   fltIntegGainFW=fltIntegGainQ;
      |   if (Idmax<0)
      |     iratio=Idmax/imax;
      |     iratio=abs(iratio);
      |     if (abs(iratio) > 1)
      |       iratio = 0;
      |     end
      |     lowlim=acos(iratio)-1.570796326794897;
      |   else
      |     lowlim=0.0;
      |   end
      |   fltLowerLimitFW=lowlim;
      |   fltUpperLimitFW=0.0;
      |   fltLambdaW=lambdaW;
      |   fltLambdaFW=lambdaFW;
      |   rampsc=polepairs*abs(ramprpm)*0.1047197551196598;
      |   fltRampUp=rampsc;
      |   fltRampDown=rampsc;
      |   fltUmaxDivImax=0.5773502691896258*udcbus/imax;
      |   if isnan(fltUmaxDivImax)
      |     if ~strcmp(fltUmaxDivImax_bkup,'0')
      |       set_param(gcb,'fltUmaxDivImax','0');
      |     end
      |   else
      |     tmps=num2str(fltUmaxDivImax);
      |     if ~strcmp(fltUmaxDivImax_bkup,tmps)
      |       set_param(gcb,'fltUmaxDivImax',tmps);
      |     end
      |   end
      |   if isnan(fltLambdaW)
      |     if ~strcmp(fltLambdaW_bkup,'0')
      |       set_param(gcb,'fltLambdaW','0');
      |     end
      |   else
      |     tmps=num2str(fltLambdaW);
      |     if ~strcmp(fltLambdaW_bkup,tmps)
      |       set_param(gcb,'fltLambdaW',tmps);
      |     end
      |   end
      |   if isnan(fltLambdaFW)
      |     if ~strcmp(fltLambdaFW_bkup,'0')
      |       set_param(gcb,'fltLambdaFW','0');
      |     end
      |   else
      |     tmps=num2str(fltLambdaFW);
      |     if ~strcmp(fltLambdaFW_bkup,tmps)
      |       set_param(gcb,'fltLambdaFW',tmps);
      |     end
      |   end
      |   if isnan(fltPropGainQ)
      |     if ~strcmp(fltPropGainQ_bkup,'0')
      |       set_param(gcb,'fltPropGainQ','0');
      |     end
      |   else
      |     tmps=num2str(fltPropGainQ);
      |     if ~strcmp(fltPropGainQ_bkup,tmps)
      |       set_param(gcb,'fltPropGainQ',tmps);
      |     end
      |   end
      |   if isnan(fltIntegGainQ)
      |     if ~strcmp(fltIntegGainQ_bkup,'0')
      |       set_param(gcb,'fltIntegGainQ','0');
      |     end
      |   else
      |     tmps=num2str(fltIntegGainQ);
      |     if ~strcmp(fltIntegGainQ_bkup,tmps)
      |       set_param(gcb,'fltIntegGainQ',tmps);
      |     end
      |   end
      |   if isnan(fltLowerLimitQ)
      |     if ~strcmp(fltLowerLimitQ_bkup,'0')
      |       set_param(gcb,'fltLowerLimitQ','0');
      |     end
      |   else
      |     tmps=num2str(fltLowerLimitQ);
      |     if ~strcmp(fltLowerLimitQ_bkup,tmps)
      |       set_param(gcb,'fltLowerLimitQ',tmps);
      |     end
      |   end
      |   if isnan(fltUpperLimitQ)
      |     if ~strcmp(fltUpperLimitQ_bkup,'0')
      |       set_param(gcb,'fltUpperLimitQ','0');
      |     end
      |   else
      |     tmps=num2str(fltUpperLimitQ);
      |     if ~strcmp(fltUpperLimitQ_bkup,tmps)
      |       set_param(gcb,'fltUpperLimitQ',tmps);
      |     end
      |   end
      |   if isnan(fltPropGainFW)
      |     if ~strcmp(fltPropGainFW_bkup,'0')
      |       set_param(gcb,'fltPropGainFW','0');
      |     end
      |   else
      |     tmps=num2str(fltPropGainFW);
      |     if ~strcmp(fltPropGainFW_bkup,tmps)
      |       set_param(gcb,'fltPropGainFW',tmps);
      |     end
      |   end
      |   if isnan(fltIntegGainFW)
      |     if ~strcmp(fltIntegGainFW_bkup,'0')
      |       set_param(gcb,'fltIntegGainFW','0');
      |     end
      |   else
      |     tmps=num2str(fltIntegGainFW);
      |     if ~strcmp(fltIntegGainFW_bkup,tmps)
      |       set_param(gcb,'fltIntegGainFW',tmps);
      |     end
      |   end
      |   if isnan(fltLowerLimitFW)
      |     if ~strcmp(fltLowerLimitFW_bkup,'0')
      |       set_param(gcb,'fltLowerLimitFW','0');
      |     end
      |   else
      |     tmps=num2str(fltLowerLimitFW);
      |     if ~strcmp(fltLowerLimitFW_bkup,tmps)
      |       set_param(gcb,'fltLowerLimitFW',tmps);
      |     end
      |   end
      |   if isnan(fltUpperLimitFW)
      |     if ~strcmp(fltUpperLimitFW_bkup,'0')
      |       set_param(gcb,'fltUpperLimitFW','0');
      |     end
      |   else
      |     tmps=num2str(fltUpperLimitFW);
      |     if ~strcmp(fltUpperLimitFW_bkup,tmps)
      |       set_param(gcb,'fltUpperLimitFW',tmps);
      |     end
      |   end
      |   if isnan(fltRampUp)
      |     if ~strcmp(fltRampUp_bkup,'0')
      |       set_param(gcb,'fltRampUp','0');
      |     end
      |   else
      |     tmps=num2str(fltRampUp);
      |     if ~strcmp(fltRampUp_bkup,tmps)
      |       set_param(gcb,'fltRampUp',tmps);
      |     end
      |   end
      |   if isnan(fltRampDown)
      |     if ~strcmp(fltRampDown_bkup,'0')
      |       set_param(gcb,'fltRampDown','0');
      |     end
      |   else
      |     tmps=num2str(fltRampDown);
      |     if ~strcmp(fltRampDown_bkup,tmps)
      |       set_param(gcb,'fltRampDown',tmps);
      |     end
      |   end
      | end
      mask Callback Idmax:
      | autoCalcEn=get_param(gcb,'autoCalcEn');
      | if strcmp(autoCalcEn,'on')
      |   SampleTime=Simulink.data.evalinGlobal(bdroot,get_param(gcb,'SampleTime'));
      |   if (SampleTime==-1)
      |     SampleTime=str2double(get_param(gcb,'SampleTime_1'));
      |   end
      |   fltUmaxDivImax_bkup=get_param(gcb,'fltUmaxDivImax');
      |   fltLambdaW_bkup=get_param(gcb,'fltLambdaW');
      |   fltLambdaFW_bkup=get_param(gcb,'fltLambdaFW');
      |   fltPropGainQ_bkup=get_param(gcb,'fltPropGainQ');
      |   fltIntegGainQ_bkup=get_param(gcb,'fltIntegGainQ');
      |   fltLowerLimitQ_bkup=get_param(gcb,'fltLowerLimitQ');
      |   fltUpperLimitQ_bkup=get_param(gcb,'fltUpperLimitQ');
      |   fltPropGainFW_bkup=get_param(gcb,'fltPropGainFW');
      |   fltIntegGainFW_bkup=get_param(gcb,'fltIntegGainFW');
      |   fltLowerLimitFW_bkup=get_param(gcb,'fltLowerLimitFW');
      |   fltUpperLimitFW_bkup=get_param(gcb,'fltUpperLimitFW');
      |   fltRampUp_bkup=get_param(gcb,'fltRampUp');
      |   fltRampDown_bkup=get_param(gcb,'fltRampDown');
      |   wf0=Simulink.data.evalinGlobal(bdroot,get_param(gcb,'wf0'));
      |   wksi=Simulink.data.evalinGlobal(bdroot,get_param(gcb,'wksi'));
      |   J=Simulink.data.evalinGlobal(bdroot,get_param(gcb,'J'));
      |   Kt=Simulink.data.evalinGlobal(bdroot,get_param(gcb,'Kt'));
      |   lambdaW=Simulink.data.evalinGlobal(bdroot,get_param(gcb,'lambdaW'));
      |   lambdaFW=Simulink.data.evalinGlobal(bdroot,get_param(gcb,'lambdaFW'));
      |   Idmax=Simulink.data.evalinGlobal(bdroot,get_param(gcb,'Idmax'));
      |   imax=Simulink.data.evalinGlobal(bdroot,get_param(gcb,'imax'));
      |   udcbus=Simulink.data.evalinGlobal(bdroot,get_param(gcb,'udcbus'));
      |   ramprpm=Simulink.data.evalinGlobal(bdroot,get_param(gcb,'ramprpm'));
      |   mechspeed=Simulink.data.evalinGlobal(bdroot,get_param(gcb,'mechspeed'));
      |   polepairs=Simulink.data.evalinGlobal(bdroot,get_param(gcb,'polepairs'));
      |   if (wf0<=0)
      |     warning('Natural frequency f0 must be positive.');
      |   end
      |   if (wksi<=0)
      |     warning('Current loop attenuation must be positive.');
      |   end
      |   if (wksi>1)
      |     warning('Current loop attenuation must not exceed 1.');
      |   end
      |   if (J<=0)
      |     warning('Moment of inertia J must be positive.');
      |   end
      |   if (Kt<=0)
      |     warning('Torque constant Kt must be positive.');
      |   end
      |   if (lambdaW<0)
      |     warning('MA filter smoothing factor must be in the range 0..1.');
      |   end
      |   if (lambdaW>1)
      |     warning('MA filter smoothing factor must be in the range 0..1.');
      |   end
      |   if (lambdaFW<0)
      |     warning('MA filter smoothing factor must be in the range 0..1.');
      |   end
      |   if (lambdaFW>1)
      |     warning('MA filter smoothing factor must be in the range 0..1.');
      |   end
      |   if (udcbus<=0)
      |     warning('DC bus voltage must be positive.');
      |   end
      |   if (imax<=0)
      |     warning('Max. phase current must be positive.');
      |   end
      |   if (mechspeed<=0)
      |     warning('Max. speed must be positive.');
      |   end
      |   if (polepairs<1)
      |     warning('Number of pole pairs must be a natural number (1, 2, 3, ...).');
      |   end
      |   if (round(polepairs)~=polepairs)
      |     warning('Number of pole pairs must be a natural number (1, 2, 3, ...).');
      |   end
      |   w0=6.283185307179586*wf0;
      |   pgain=2.0*wksi*w0*J/Kt;
      |   igain=w0*w0*J/Kt;
      |   wmax=polepairs*mechspeed*0.1047197551196598;
      |   fltPropGainQ=pgain;
      |   fltIntegGainQ=igain*SampleTime*0.5;
      |   fltLowerLimitQ=-wmax;
      |   fltUpperLimitQ=wmax;
      |   fltPropGainFW=0.9*pgain;
      |   fltIntegGainFW=fltIntegGainQ;
      |   if (Idmax<0)
      |     iratio=Idmax/imax;
      |     iratio=abs(iratio);
      |     if (abs(iratio) > 1)
      |       iratio = 0;
      |     end
      |     lowlim=acos(iratio)-1.570796326794897;
      |   else
      |     lowlim=0.0;
      |   end
      |   fltLowerLimitFW=lowlim;
      |   fltUpperLimitFW=0.0;
      |   fltLambdaW=lambdaW;
      |   fltLambdaFW=lambdaFW;
      |   rampsc=polepairs*abs(ramprpm)*0.1047197551196598;
      |   fltRampUp=rampsc;
      |   fltRampDown=rampsc;
      |   fltUmaxDivImax=0.5773502691896258*udcbus/imax;
      |   if isnan(fltUmaxDivImax)
      |     if ~strcmp(fltUmaxDivImax_bkup,'0')
      |       set_param(gcb,'fltUmaxDivImax','0');
      |     end
      |   else
      |     tmps=num2str(fltUmaxDivImax);
      |     if ~strcmp(fltUmaxDivImax_bkup,tmps)
      |       set_param(gcb,'fltUmaxDivImax',tmps);
      |     end
      |   end
      |   if isnan(fltLambdaW)
      |     if ~strcmp(fltLambdaW_bkup,'0')
      |       set_param(gcb,'fltLambdaW','0');
      |     end
      |   else
      |     tmps=num2str(fltLambdaW);
      |     if ~strcmp(fltLambdaW_bkup,tmps)
      |       set_param(gcb,'fltLambdaW',tmps);
      |     end
      |   end
      |   if isnan(fltLambdaFW)
      |     if ~strcmp(fltLambdaFW_bkup,'0')
      |       set_param(gcb,'fltLambdaFW','0');
      |     end
      |   else
      |     tmps=num2str(fltLambdaFW);
      |     if ~strcmp(fltLambdaFW_bkup,tmps)
      |       set_param(gcb,'fltLambdaFW',tmps);
      |     end
      |   end
      |   if isnan(fltPropGainQ)
      |     if ~strcmp(fltPropGainQ_bkup,'0')
      |       set_param(gcb,'fltPropGainQ','0');
      |     end
      |   else
      |     tmps=num2str(fltPropGainQ);
      |     if ~strcmp(fltPropGainQ_bkup,tmps)
      |       set_param(gcb,'fltPropGainQ',tmps);
      |     end
      |   end
      |   if isnan(fltIntegGainQ)
      |     if ~strcmp(fltIntegGainQ_bkup,'0')
      |       set_param(gcb,'fltIntegGainQ','0');
      |     end
      |   else
      |     tmps=num2str(fltIntegGainQ);
      |     if ~strcmp(fltIntegGainQ_bkup,tmps)
      |       set_param(gcb,'fltIntegGainQ',tmps);
      |     end
      |   end
      |   if isnan(fltLowerLimitQ)
      |     if ~strcmp(fltLowerLimitQ_bkup,'0')
      |       set_param(gcb,'fltLowerLimitQ','0');
      |     end
      |   else
      |     tmps=num2str(fltLowerLimitQ);
      |     if ~strcmp(fltLowerLimitQ_bkup,tmps)
      |       set_param(gcb,'fltLowerLimitQ',tmps);
      |     end
      |   end
      |   if isnan(fltUpperLimitQ)
      |     if ~strcmp(fltUpperLimitQ_bkup,'0')
      |       set_param(gcb,'fltUpperLimitQ','0');
      |     end
      |   else
      |     tmps=num2str(fltUpperLimitQ);
      |     if ~strcmp(fltUpperLimitQ_bkup,tmps)
      |       set_param(gcb,'fltUpperLimitQ',tmps);
      |     end
      |   end
      |   if isnan(fltPropGainFW)
      |     if ~strcmp(fltPropGainFW_bkup,'0')
      |       set_param(gcb,'fltPropGainFW','0');
      |     end
      |   else
      |     tmps=num2str(fltPropGainFW);
      |     if ~strcmp(fltPropGainFW_bkup,tmps)
      |       set_param(gcb,'fltPropGainFW',tmps);
      |     end
      |   end
      |   if isnan(fltIntegGainFW)
      |     if ~strcmp(fltIntegGainFW_bkup,'0')
      |       set_param(gcb,'fltIntegGainFW','0');
      |     end
      |   else
      |     tmps=num2str(fltIntegGainFW);
      |     if ~strcmp(fltIntegGainFW_bkup,tmps)
      |       set_param(gcb,'fltIntegGainFW',tmps);
      |     end
      |   end
      |   if isnan(fltLowerLimitFW)
      |     if ~strcmp(fltLowerLimitFW_bkup,'0')
      |       set_param(gcb,'fltLowerLimitFW','0');
      |     end
      |   else
      |     tmps=num2str(fltLowerLimitFW);
      |     if ~strcmp(fltLowerLimitFW_bkup,tmps)
      |       set_param(gcb,'fltLowerLimitFW',tmps);
      |     end
      |   end
      |   if isnan(fltUpperLimitFW)
      |     if ~strcmp(fltUpperLimitFW_bkup,'0')
      |       set_param(gcb,'fltUpperLimitFW','0');
      |     end
      |   else
      |     tmps=num2str(fltUpperLimitFW);
      |     if ~strcmp(fltUpperLimitFW_bkup,tmps)
      |       set_param(gcb,'fltUpperLimitFW',tmps);
      |     end
      |   end
      |   if isnan(fltRampUp)
      |     if ~strcmp(fltRampUp_bkup,'0')
      |       set_param(gcb,'fltRampUp','0');
      |     end
      |   else
      |     tmps=num2str(fltRampUp);
      |     if ~strcmp(fltRampUp_bkup,tmps)
      |       set_param(gcb,'fltRampUp',tmps);
      |     end
      |   end
      |   if isnan(fltRampDown)
      |     if ~strcmp(fltRampDown_bkup,'0')
      |       set_param(gcb,'fltRampDown','0');
      |     end
      |   else
      |     tmps=num2str(fltRampDown);
      |     if ~strcmp(fltRampDown_bkup,tmps)
      |       set_param(gcb,'fltRampDown',tmps);
      |     end
      |   end
      | end
      mask Callback imax:
      | autoCalcEn=get_param(gcb,'autoCalcEn');
      | if strcmp(autoCalcEn,'on')
      |   SampleTime=Simulink.data.evalinGlobal(bdroot,get_param(gcb,'SampleTime'));
      |   if (SampleTime==-1)
      |     SampleTime=str2double(get_param(gcb,'SampleTime_1'));
      |   end
      |   fltUmaxDivImax_bkup=get_param(gcb,'fltUmaxDivImax');
      |   fltLambdaW_bkup=get_param(gcb,'fltLambdaW');
      |   fltLambdaFW_bkup=get_param(gcb,'fltLambdaFW');
      |   fltPropGainQ_bkup=get_param(gcb,'fltPropGainQ');
      |   fltIntegGainQ_bkup=get_param(gcb,'fltIntegGainQ');
      |   fltLowerLimitQ_bkup=get_param(gcb,'fltLowerLimitQ');
      |   fltUpperLimitQ_bkup=get_param(gcb,'fltUpperLimitQ');
      |   fltPropGainFW_bkup=get_param(gcb,'fltPropGainFW');
      |   fltIntegGainFW_bkup=get_param(gcb,'fltIntegGainFW');
      |   fltLowerLimitFW_bkup=get_param(gcb,'fltLowerLimitFW');
      |   fltUpperLimitFW_bkup=get_param(gcb,'fltUpperLimitFW');
      |   fltRampUp_bkup=get_param(gcb,'fltRampUp');
      |   fltRampDown_bkup=get_param(gcb,'fltRampDown');
      |   wf0=Simulink.data.evalinGlobal(bdroot,get_param(gcb,'wf0'));
      |   wksi=Simulink.data.evalinGlobal(bdroot,get_param(gcb,'wksi'));
      |   J=Simulink.data.evalinGlobal(bdroot,get_param(gcb,'J'));
      |   Kt=Simulink.data.evalinGlobal(bdroot,get_param(gcb,'Kt'));
      |   lambdaW=Simulink.data.evalinGlobal(bdroot,get_param(gcb,'lambdaW'));
      |   lambdaFW=Simulink.data.evalinGlobal(bdroot,get_param(gcb,'lambdaFW'));
      |   Idmax=Simulink.data.evalinGlobal(bdroot,get_param(gcb,'Idmax'));
      |   imax=Simulink.data.evalinGlobal(bdroot,get_param(gcb,'imax'));
      |   udcbus=Simulink.data.evalinGlobal(bdroot,get_param(gcb,'udcbus'));
      |   ramprpm=Simulink.data.evalinGlobal(bdroot,get_param(gcb,'ramprpm'));
      |   mechspeed=Simulink.data.evalinGlobal(bdroot,get_param(gcb,'mechspeed'));
      |   polepairs=Simulink.data.evalinGlobal(bdroot,get_param(gcb,'polepairs'));
      |   if (wf0<=0)
      |     warning('Natural frequency f0 must be positive.');
      |   end
      |   if (wksi<=0)
      |     warning('Current loop attenuation must be positive.');
      |   end
      |   if (wksi>1)
      |     warning('Current loop attenuation must not exceed 1.');
      |   end
      |   if (J<=0)
      |     warning('Moment of inertia J must be positive.');
      |   end
      |   if (Kt<=0)
      |     warning('Torque constant Kt must be positive.');
      |   end
      |   if (lambdaW<0)
      |     warning('MA filter smoothing factor must be in the range 0..1.');
      |   end
      |   if (lambdaW>1)
      |     warning('MA filter smoothing factor must be in the range 0..1.');
      |   end
      |   if (lambdaFW<0)
      |     warning('MA filter smoothing factor must be in the range 0..1.');
      |   end
      |   if (lambdaFW>1)
      |     warning('MA filter smoothing factor must be in the range 0..1.');
      |   end
      |   if (udcbus<=0)
      |     warning('DC bus voltage must be positive.');
      |   end
      |   if (imax<=0)
      |     warning('Max. phase current must be positive.');
      |   end
      |   if (mechspeed<=0)
      |     warning('Max. speed must be positive.');
      |   end
      |   if (polepairs<1)
      |     warning('Number of pole pairs must be a natural number (1, 2, 3, ...).');
      |   end
      |   if (round(polepairs)~=polepairs)
      |     warning('Number of pole pairs must be a natural number (1, 2, 3, ...).');
      |   end
      |   w0=6.283185307179586*wf0;
      |   pgain=2.0*wksi*w0*J/Kt;
      |   igain=w0*w0*J/Kt;
      |   wmax=polepairs*mechspeed*0.1047197551196598;
      |   fltPropGainQ=pgain;
      |   fltIntegGainQ=igain*SampleTime*0.5;
      |   fltLowerLimitQ=-wmax;
      |   fltUpperLimitQ=wmax;
      |   fltPropGainFW=0.9*pgain;
      |   fltIntegGainFW=fltIntegGainQ;
      |   if (Idmax<0)
      |     iratio=Idmax/imax;
      |     iratio=abs(iratio);
      |     if (abs(iratio) > 1)
      |       iratio = 0;
      |     end
      |     lowlim=acos(iratio)-1.570796326794897;
      |   else
      |     lowlim=0.0;
      |   end
      |   fltLowerLimitFW=lowlim;
      |   fltUpperLimitFW=0.0;
      |   fltLambdaW=lambdaW;
      |   fltLambdaFW=lambdaFW;
      |   rampsc=polepairs*abs(ramprpm)*0.1047197551196598;
      |   fltRampUp=rampsc;
      |   fltRampDown=rampsc;
      |   fltUmaxDivImax=0.5773502691896258*udcbus/imax;
      |   if isnan(fltUmaxDivImax)
      |     if ~strcmp(fltUmaxDivImax_bkup,'0')
      |       set_param(gcb,'fltUmaxDivImax','0');
      |     end
      |   else
      |     tmps=num2str(fltUmaxDivImax);
      |     if ~strcmp(fltUmaxDivImax_bkup,tmps)
      |       set_param(gcb,'fltUmaxDivImax',tmps);
      |     end
      |   end
      |   if isnan(fltLambdaW)
      |     if ~strcmp(fltLambdaW_bkup,'0')
      |       set_param(gcb,'fltLambdaW','0');
      |     end
      |   else
      |     tmps=num2str(fltLambdaW);
      |     if ~strcmp(fltLambdaW_bkup,tmps)
      |       set_param(gcb,'fltLambdaW',tmps);
      |     end
      |   end
      |   if isnan(fltLambdaFW)
      |     if ~strcmp(fltLambdaFW_bkup,'0')
      |       set_param(gcb,'fltLambdaFW','0');
      |     end
      |   else
      |     tmps=num2str(fltLambdaFW);
      |     if ~strcmp(fltLambdaFW_bkup,tmps)
      |       set_param(gcb,'fltLambdaFW',tmps);
      |     end
      |   end
      |   if isnan(fltPropGainQ)
      |     if ~strcmp(fltPropGainQ_bkup,'0')
      |       set_param(gcb,'fltPropGainQ','0');
      |     end
      |   else
      |     tmps=num2str(fltPropGainQ);
      |     if ~strcmp(fltPropGainQ_bkup,tmps)
      |       set_param(gcb,'fltPropGainQ',tmps);
      |     end
      |   end
      |   if isnan(fltIntegGainQ)
      |     if ~strcmp(fltIntegGainQ_bkup,'0')
      |       set_param(gcb,'fltIntegGainQ','0');
      |     end
      |   else
      |     tmps=num2str(fltIntegGainQ);
      |     if ~strcmp(fltIntegGainQ_bkup,tmps)
      |       set_param(gcb,'fltIntegGainQ',tmps);
      |     end
      |   end
      |   if isnan(fltLowerLimitQ)
      |     if ~strcmp(fltLowerLimitQ_bkup,'0')
      |       set_param(gcb,'fltLowerLimitQ','0');
      |     end
      |   else
      |     tmps=num2str(fltLowerLimitQ);
      |     if ~strcmp(fltLowerLimitQ_bkup,tmps)
      |       set_param(gcb,'fltLowerLimitQ',tmps);
      |     end
      |   end
      |   if isnan(fltUpperLimitQ)
      |     if ~strcmp(fltUpperLimitQ_bkup,'0')
      |       set_param(gcb,'fltUpperLimitQ','0');
      |     end
      |   else
      |     tmps=num2str(fltUpperLimitQ);
      |     if ~strcmp(fltUpperLimitQ_bkup,tmps)
      |       set_param(gcb,'fltUpperLimitQ',tmps);
      |     end
      |   end
      |   if isnan(fltPropGainFW)
      |     if ~strcmp(fltPropGainFW_bkup,'0')
      |       set_param(gcb,'fltPropGainFW','0');
      |     end
      |   else
      |     tmps=num2str(fltPropGainFW);
      |     if ~strcmp(fltPropGainFW_bkup,tmps)
      |       set_param(gcb,'fltPropGainFW',tmps);
      |     end
      |   end
      |   if isnan(fltIntegGainFW)
      |     if ~strcmp(fltIntegGainFW_bkup,'0')
      |       set_param(gcb,'fltIntegGainFW','0');
      |     end
      |   else
      |     tmps=num2str(fltIntegGainFW);
      |     if ~strcmp(fltIntegGainFW_bkup,tmps)
      |       set_param(gcb,'fltIntegGainFW',tmps);
      |     end
      |   end
      |   if isnan(fltLowerLimitFW)
      |     if ~strcmp(fltLowerLimitFW_bkup,'0')
      |       set_param(gcb,'fltLowerLimitFW','0');
      |     end
      |   else
      |     tmps=num2str(fltLowerLimitFW);
      |     if ~strcmp(fltLowerLimitFW_bkup,tmps)
      |       set_param(gcb,'fltLowerLimitFW',tmps);
      |     end
      |   end
      |   if isnan(fltUpperLimitFW)
      |     if ~strcmp(fltUpperLimitFW_bkup,'0')
      |       set_param(gcb,'fltUpperLimitFW','0');
      |     end
      |   else
      |     tmps=num2str(fltUpperLimitFW);
      |     if ~strcmp(fltUpperLimitFW_bkup,tmps)
      |       set_param(gcb,'fltUpperLimitFW',tmps);
      |     end
      |   end
      |   if isnan(fltRampUp)
      |     if ~strcmp(fltRampUp_bkup,'0')
      |       set_param(gcb,'fltRampUp','0');
      |     end
      |   else
      |     tmps=num2str(fltRampUp);
      |     if ~strcmp(fltRampUp_bkup,tmps)
      |       set_param(gcb,'fltRampUp',tmps);
      |     end
      |   end
      |   if isnan(fltRampDown)
      |     if ~strcmp(fltRampDown_bkup,'0')
      |       set_param(gcb,'fltRampDown','0');
      |     end
      |   else
      |     tmps=num2str(fltRampDown);
      |     if ~strcmp(fltRampDown_bkup,tmps)
      |       set_param(gcb,'fltRampDown',tmps);
      |     end
      |   end
      | end
      mask Callback udcbus:
      | autoCalcEn=get_param(gcb,'autoCalcEn');
      | if strcmp(autoCalcEn,'on')
      |   SampleTime=Simulink.data.evalinGlobal(bdroot,get_param(gcb,'SampleTime'));
      |   if (SampleTime==-1)
      |     SampleTime=str2double(get_param(gcb,'SampleTime_1'));
      |   end
      |   fltUmaxDivImax_bkup=get_param(gcb,'fltUmaxDivImax');
      |   fltLambdaW_bkup=get_param(gcb,'fltLambdaW');
      |   fltLambdaFW_bkup=get_param(gcb,'fltLambdaFW');
      |   fltPropGainQ_bkup=get_param(gcb,'fltPropGainQ');
      |   fltIntegGainQ_bkup=get_param(gcb,'fltIntegGainQ');
      |   fltLowerLimitQ_bkup=get_param(gcb,'fltLowerLimitQ');
      |   fltUpperLimitQ_bkup=get_param(gcb,'fltUpperLimitQ');
      |   fltPropGainFW_bkup=get_param(gcb,'fltPropGainFW');
      |   fltIntegGainFW_bkup=get_param(gcb,'fltIntegGainFW');
      |   fltLowerLimitFW_bkup=get_param(gcb,'fltLowerLimitFW');
      |   fltUpperLimitFW_bkup=get_param(gcb,'fltUpperLimitFW');
      |   fltRampUp_bkup=get_param(gcb,'fltRampUp');
      |   fltRampDown_bkup=get_param(gcb,'fltRampDown');
      |   wf0=Simulink.data.evalinGlobal(bdroot,get_param(gcb,'wf0'));
      |   wksi=Simulink.data.evalinGlobal(bdroot,get_param(gcb,'wksi'));
      |   J=Simulink.data.evalinGlobal(bdroot,get_param(gcb,'J'));
      |   Kt=Simulink.data.evalinGlobal(bdroot,get_param(gcb,'Kt'));
      |   lambdaW=Simulink.data.evalinGlobal(bdroot,get_param(gcb,'lambdaW'));
      |   lambdaFW=Simulink.data.evalinGlobal(bdroot,get_param(gcb,'lambdaFW'));
      |   Idmax=Simulink.data.evalinGlobal(bdroot,get_param(gcb,'Idmax'));
      |   imax=Simulink.data.evalinGlobal(bdroot,get_param(gcb,'imax'));
      |   udcbus=Simulink.data.evalinGlobal(bdroot,get_param(gcb,'udcbus'));
      |   ramprpm=Simulink.data.evalinGlobal(bdroot,get_param(gcb,'ramprpm'));
      |   mechspeed=Simulink.data.evalinGlobal(bdroot,get_param(gcb,'mechspeed'));
      |   polepairs=Simulink.data.evalinGlobal(bdroot,get_param(gcb,'polepairs'));
      |   if (wf0<=0)
      |     warning('Natural frequency f0 must be positive.');
      |   end
      |   if (wksi<=0)
      |     warning('Current loop attenuation must be positive.');
      |   end
      |   if (wksi>1)
      |     warning('Current loop attenuation must not exceed 1.');
      |   end
      |   if (J<=0)
      |     warning('Moment of inertia J must be positive.');
      |   end
      |   if (Kt<=0)
      |     warning('Torque constant Kt must be positive.');
      |   end
      |   if (lambdaW<0)
      |     warning('MA filter smoothing factor must be in the range 0..1.');
      |   end
      |   if (lambdaW>1)
      |     warning('MA filter smoothing factor must be in the range 0..1.');
      |   end
      |   if (lambdaFW<0)
      |     warning('MA filter smoothing factor must be in the range 0..1.');
      |   end
      |   if (lambdaFW>1)
      |     warning('MA filter smoothing factor must be in the range 0..1.');
      |   end
      |   if (udcbus<=0)
      |     warning('DC bus voltage must be positive.');
      |   end
      |   if (imax<=0)
      |     warning('Max. phase current must be positive.');
      |   end
      |   if (mechspeed<=0)
      |     warning('Max. speed must be positive.');
      |   end
      |   if (polepairs<1)
      |     warning('Number of pole pairs must be a natural number (1, 2, 3, ...).');
      |   end
      |   if (round(polepairs)~=polepairs)
      |     warning('Number of pole pairs must be a natural number (1, 2, 3, ...).');
      |   end
      |   w0=6.283185307179586*wf0;
      |   pgain=2.0*wksi*w0*J/Kt;
      |   igain=w0*w0*J/Kt;
      |   wmax=polepairs*mechspeed*0.1047197551196598;
      |   fltPropGainQ=pgain;
      |   fltIntegGainQ=igain*SampleTime*0.5;
      |   fltLowerLimitQ=-wmax;
      |   fltUpperLimitQ=wmax;
      |   fltPropGainFW=0.9*pgain;
      |   fltIntegGainFW=fltIntegGainQ;
      |   if (Idmax<0)
      |     iratio=Idmax/imax;
      |     iratio=abs(iratio);
      |     if (abs(iratio) > 1)
      |       iratio = 0;
      |     end
      |     lowlim=acos(iratio)-1.570796326794897;
      |   else
      |     lowlim=0.0;
      |   end
      |   fltLowerLimitFW=lowlim;
      |   fltUpperLimitFW=0.0;
      |   fltLambdaW=lambdaW;
      |   fltLambdaFW=lambdaFW;
      |   rampsc=polepairs*abs(ramprpm)*0.1047197551196598;
      |   fltRampUp=rampsc;
      |   fltRampDown=rampsc;
      |   fltUmaxDivImax=0.5773502691896258*udcbus/imax;
      |   if isnan(fltUmaxDivImax)
      |     if ~strcmp(fltUmaxDivImax_bkup,'0')
      |       set_param(gcb,'fltUmaxDivImax','0');
      |     end
      |   else
      |     tmps=num2str(fltUmaxDivImax);
      |     if ~strcmp(fltUmaxDivImax_bkup,tmps)
      |       set_param(gcb,'fltUmaxDivImax',tmps);
      |     end
      |   end
      |   if isnan(fltLambdaW)
      |     if ~strcmp(fltLambdaW_bkup,'0')
      |       set_param(gcb,'fltLambdaW','0');
      |     end
      |   else
      |     tmps=num2str(fltLambdaW);
      |     if ~strcmp(fltLambdaW_bkup,tmps)
      |       set_param(gcb,'fltLambdaW',tmps);
      |     end
      |   end
      |   if isnan(fltLambdaFW)
      |     if ~strcmp(fltLambdaFW_bkup,'0')
      |       set_param(gcb,'fltLambdaFW','0');
      |     end
      |   else
      |     tmps=num2str(fltLambdaFW);
      |     if ~strcmp(fltLambdaFW_bkup,tmps)
      |       set_param(gcb,'fltLambdaFW',tmps);
      |     end
      |   end
      |   if isnan(fltPropGainQ)
      |     if ~strcmp(fltPropGainQ_bkup,'0')
      |       set_param(gcb,'fltPropGainQ','0');
      |     end
      |   else
      |     tmps=num2str(fltPropGainQ);
      |     if ~strcmp(fltPropGainQ_bkup,tmps)
      |       set_param(gcb,'fltPropGainQ',tmps);
      |     end
      |   end
      |   if isnan(fltIntegGainQ)
      |     if ~strcmp(fltIntegGainQ_bkup,'0')
      |       set_param(gcb,'fltIntegGainQ','0');
      |     end
      |   else
      |     tmps=num2str(fltIntegGainQ);
      |     if ~strcmp(fltIntegGainQ_bkup,tmps)
      |       set_param(gcb,'fltIntegGainQ',tmps);
      |     end
      |   end
      |   if isnan(fltLowerLimitQ)
      |     if ~strcmp(fltLowerLimitQ_bkup,'0')
      |       set_param(gcb,'fltLowerLimitQ','0');
      |     end
      |   else
      |     tmps=num2str(fltLowerLimitQ);
      |     if ~strcmp(fltLowerLimitQ_bkup,tmps)
      |       set_param(gcb,'fltLowerLimitQ',tmps);
      |     end
      |   end
      |   if isnan(fltUpperLimitQ)
      |     if ~strcmp(fltUpperLimitQ_bkup,'0')
      |       set_param(gcb,'fltUpperLimitQ','0');
      |     end
      |   else
      |     tmps=num2str(fltUpperLimitQ);
      |     if ~strcmp(fltUpperLimitQ_bkup,tmps)
      |       set_param(gcb,'fltUpperLimitQ',tmps);
      |     end
      |   end
      |   if isnan(fltPropGainFW)
      |     if ~strcmp(fltPropGainFW_bkup,'0')
      |       set_param(gcb,'fltPropGainFW','0');
      |     end
      |   else
      |     tmps=num2str(fltPropGainFW);
      |     if ~strcmp(fltPropGainFW_bkup,tmps)
      |       set_param(gcb,'fltPropGainFW',tmps);
      |     end
      |   end
      |   if isnan(fltIntegGainFW)
      |     if ~strcmp(fltIntegGainFW_bkup,'0')
      |       set_param(gcb,'fltIntegGainFW','0');
      |     end
      |   else
      |     tmps=num2str(fltIntegGainFW);
      |     if ~strcmp(fltIntegGainFW_bkup,tmps)
      |       set_param(gcb,'fltIntegGainFW',tmps);
      |     end
      |   end
      |   if isnan(fltLowerLimitFW)
      |     if ~strcmp(fltLowerLimitFW_bkup,'0')
      |       set_param(gcb,'fltLowerLimitFW','0');
      |     end
      |   else
      |     tmps=num2str(fltLowerLimitFW);
      |     if ~strcmp(fltLowerLimitFW_bkup,tmps)
      |       set_param(gcb,'fltLowerLimitFW',tmps);
      |     end
      |   end
      |   if isnan(fltUpperLimitFW)
      |     if ~strcmp(fltUpperLimitFW_bkup,'0')
      |       set_param(gcb,'fltUpperLimitFW','0');
      |     end
      |   else
      |     tmps=num2str(fltUpperLimitFW);
      |     if ~strcmp(fltUpperLimitFW_bkup,tmps)
      |       set_param(gcb,'fltUpperLimitFW',tmps);
      |     end
      |   end
      |   if isnan(fltRampUp)
      |     if ~strcmp(fltRampUp_bkup,'0')
      |       set_param(gcb,'fltRampUp','0');
      |     end
      |   else
      |     tmps=num2str(fltRampUp);
      |     if ~strcmp(fltRampUp_bkup,tmps)
      |       set_param(gcb,'fltRampUp',tmps);
      |     end
      |   end
      |   if isnan(fltRampDown)
      |     if ~strcmp(fltRampDown_bkup,'0')
      |       set_param(gcb,'fltRampDown','0');
      |     end
      |   else
      |     tmps=num2str(fltRampDown);
      |     if ~strcmp(fltRampDown_bkup,tmps)
      |       set_param(gcb,'fltRampDown',tmps);
      |     end
      |   end
      | end
      mask Callback ramprpm:
      | autoCalcEn=get_param(gcb,'autoCalcEn');
      | if strcmp(autoCalcEn,'on')
      |   SampleTime=Simulink.data.evalinGlobal(bdroot,get_param(gcb,'SampleTime'));
      |   if (SampleTime==-1)
      |     SampleTime=str2double(get_param(gcb,'SampleTime_1'));
      |   end
      |   fltUmaxDivImax_bkup=get_param(gcb,'fltUmaxDivImax');
      |   fltLambdaW_bkup=get_param(gcb,'fltLambdaW');
      |   fltLambdaFW_bkup=get_param(gcb,'fltLambdaFW');
      |   fltPropGainQ_bkup=get_param(gcb,'fltPropGainQ');
      |   fltIntegGainQ_bkup=get_param(gcb,'fltIntegGainQ');
      |   fltLowerLimitQ_bkup=get_param(gcb,'fltLowerLimitQ');
      |   fltUpperLimitQ_bkup=get_param(gcb,'fltUpperLimitQ');
      |   fltPropGainFW_bkup=get_param(gcb,'fltPropGainFW');
      |   fltIntegGainFW_bkup=get_param(gcb,'fltIntegGainFW');
      |   fltLowerLimitFW_bkup=get_param(gcb,'fltLowerLimitFW');
      |   fltUpperLimitFW_bkup=get_param(gcb,'fltUpperLimitFW');
      |   fltRampUp_bkup=get_param(gcb,'fltRampUp');
      |   fltRampDown_bkup=get_param(gcb,'fltRampDown');
      |   wf0=Simulink.data.evalinGlobal(bdroot,get_param(gcb,'wf0'));
      |   wksi=Simulink.data.evalinGlobal(bdroot,get_param(gcb,'wksi'));
      |   J=Simulink.data.evalinGlobal(bdroot,get_param(gcb,'J'));
      |   Kt=Simulink.data.evalinGlobal(bdroot,get_param(gcb,'Kt'));
      |   lambdaW=Simulink.data.evalinGlobal(bdroot,get_param(gcb,'lambdaW'));
      |   lambdaFW=Simulink.data.evalinGlobal(bdroot,get_param(gcb,'lambdaFW'));
      |   Idmax=Simulink.data.evalinGlobal(bdroot,get_param(gcb,'Idmax'));
      |   imax=Simulink.data.evalinGlobal(bdroot,get_param(gcb,'imax'));
      |   udcbus=Simulink.data.evalinGlobal(bdroot,get_param(gcb,'udcbus'));
      |   ramprpm=Simulink.data.evalinGlobal(bdroot,get_param(gcb,'ramprpm'));
      |   mechspeed=Simulink.data.evalinGlobal(bdroot,get_param(gcb,'mechspeed'));
      |   polepairs=Simulink.data.evalinGlobal(bdroot,get_param(gcb,'polepairs'));
      |   if (wf0<=0)
      |     warning('Natural frequency f0 must be positive.');
      |   end
      |   if (wksi<=0)
      |     warning('Current loop attenuation must be positive.');
      |   end
      |   if (wksi>1)
      |     warning('Current loop attenuation must not exceed 1.');
      |   end
      |   if (J<=0)
      |     warning('Moment of inertia J must be positive.');
      |   end
      |   if (Kt<=0)
      |     warning('Torque constant Kt must be positive.');
      |   end
      |   if (lambdaW<0)
      |     warning('MA filter smoothing factor must be in the range 0..1.');
      |   end
      |   if (lambdaW>1)
      |     warning('MA filter smoothing factor must be in the range 0..1.');
      |   end
      |   if (lambdaFW<0)
      |     warning('MA filter smoothing factor must be in the range 0..1.');
      |   end
      |   if (lambdaFW>1)
      |     warning('MA filter smoothing factor must be in the range 0..1.');
      |   end
      |   if (udcbus<=0)
      |     warning('DC bus voltage must be positive.');
      |   end
      |   if (imax<=0)
      |     warning('Max. phase current must be positive.');
      |   end
      |   if (mechspeed<=0)
      |     warning('Max. speed must be positive.');
      |   end
      |   if (polepairs<1)
      |     warning('Number of pole pairs must be a natural number (1, 2, 3, ...).');
      |   end
      |   if (round(polepairs)~=polepairs)
      |     warning('Number of pole pairs must be a natural number (1, 2, 3, ...).');
      |   end
      |   w0=6.283185307179586*wf0;
      |   pgain=2.0*wksi*w0*J/Kt;
      |   igain=w0*w0*J/Kt;
      |   wmax=polepairs*mechspeed*0.1047197551196598;
      |   fltPropGainQ=pgain;
      |   fltIntegGainQ=igain*SampleTime*0.5;
      |   fltLowerLimitQ=-wmax;
      |   fltUpperLimitQ=wmax;
      |   fltPropGainFW=0.9*pgain;
      |   fltIntegGainFW=fltIntegGainQ;
      |   if (Idmax<0)
      |     iratio=Idmax/imax;
      |     iratio=abs(iratio);
      |     if (abs(iratio) > 1)
      |       iratio = 0;
      |     end
      |     lowlim=acos(iratio)-1.570796326794897;
      |   else
      |     lowlim=0.0;
      |   end
      |   fltLowerLimitFW=lowlim;
      |   fltUpperLimitFW=0.0;
      |   fltLambdaW=lambdaW;
      |   fltLambdaFW=lambdaFW;
      |   rampsc=polepairs*abs(ramprpm)*0.1047197551196598;
      |   fltRampUp=rampsc;
      |   fltRampDown=rampsc;
      |   fltUmaxDivImax=0.5773502691896258*udcbus/imax;
      |   if isnan(fltUmaxDivImax)
      |     if ~strcmp(fltUmaxDivImax_bkup,'0')
      |       set_param(gcb,'fltUmaxDivImax','0');
      |     end
      |   else
      |     tmps=num2str(fltUmaxDivImax);
      |     if ~strcmp(fltUmaxDivImax_bkup,tmps)
      |       set_param(gcb,'fltUmaxDivImax',tmps);
      |     end
      |   end
      |   if isnan(fltLambdaW)
      |     if ~strcmp(fltLambdaW_bkup,'0')
      |       set_param(gcb,'fltLambdaW','0');
      |     end
      |   else
      |     tmps=num2str(fltLambdaW);
      |     if ~strcmp(fltLambdaW_bkup,tmps)
      |       set_param(gcb,'fltLambdaW',tmps);
      |     end
      |   end
      |   if isnan(fltLambdaFW)
      |     if ~strcmp(fltLambdaFW_bkup,'0')
      |       set_param(gcb,'fltLambdaFW','0');
      |     end
      |   else
      |     tmps=num2str(fltLambdaFW);
      |     if ~strcmp(fltLambdaFW_bkup,tmps)
      |       set_param(gcb,'fltLambdaFW',tmps);
      |     end
      |   end
      |   if isnan(fltPropGainQ)
      |     if ~strcmp(fltPropGainQ_bkup,'0')
      |       set_param(gcb,'fltPropGainQ','0');
      |     end
      |   else
      |     tmps=num2str(fltPropGainQ);
      |     if ~strcmp(fltPropGainQ_bkup,tmps)
      |       set_param(gcb,'fltPropGainQ',tmps);
      |     end
      |   end
      |   if isnan(fltIntegGainQ)
      |     if ~strcmp(fltIntegGainQ_bkup,'0')
      |       set_param(gcb,'fltIntegGainQ','0');
      |     end
      |   else
      |     tmps=num2str(fltIntegGainQ);
      |     if ~strcmp(fltIntegGainQ_bkup,tmps)
      |       set_param(gcb,'fltIntegGainQ',tmps);
      |     end
      |   end
      |   if isnan(fltLowerLimitQ)
      |     if ~strcmp(fltLowerLimitQ_bkup,'0')
      |       set_param(gcb,'fltLowerLimitQ','0');
      |     end
      |   else
      |     tmps=num2str(fltLowerLimitQ);
      |     if ~strcmp(fltLowerLimitQ_bkup,tmps)
      |       set_param(gcb,'fltLowerLimitQ',tmps);
      |     end
      |   end
      |   if isnan(fltUpperLimitQ)
      |     if ~strcmp(fltUpperLimitQ_bkup,'0')
      |       set_param(gcb,'fltUpperLimitQ','0');
      |     end
      |   else
      |     tmps=num2str(fltUpperLimitQ);
      |     if ~strcmp(fltUpperLimitQ_bkup,tmps)
      |       set_param(gcb,'fltUpperLimitQ',tmps);
      |     end
      |   end
      |   if isnan(fltPropGainFW)
      |     if ~strcmp(fltPropGainFW_bkup,'0')
      |       set_param(gcb,'fltPropGainFW','0');
      |     end
      |   else
      |     tmps=num2str(fltPropGainFW);
      |     if ~strcmp(fltPropGainFW_bkup,tmps)
      |       set_param(gcb,'fltPropGainFW',tmps);
      |     end
      |   end
      |   if isnan(fltIntegGainFW)
      |     if ~strcmp(fltIntegGainFW_bkup,'0')
      |       set_param(gcb,'fltIntegGainFW','0');
      |     end
      |   else
      |     tmps=num2str(fltIntegGainFW);
      |     if ~strcmp(fltIntegGainFW_bkup,tmps)
      |       set_param(gcb,'fltIntegGainFW',tmps);
      |     end
      |   end
      |   if isnan(fltLowerLimitFW)
      |     if ~strcmp(fltLowerLimitFW_bkup,'0')
      |       set_param(gcb,'fltLowerLimitFW','0');
      |     end
      |   else
      |     tmps=num2str(fltLowerLimitFW);
      |     if ~strcmp(fltLowerLimitFW_bkup,tmps)
      |       set_param(gcb,'fltLowerLimitFW',tmps);
      |     end
      |   end
      |   if isnan(fltUpperLimitFW)
      |     if ~strcmp(fltUpperLimitFW_bkup,'0')
      |       set_param(gcb,'fltUpperLimitFW','0');
      |     end
      |   else
      |     tmps=num2str(fltUpperLimitFW);
      |     if ~strcmp(fltUpperLimitFW_bkup,tmps)
      |       set_param(gcb,'fltUpperLimitFW',tmps);
      |     end
      |   end
      |   if isnan(fltRampUp)
      |     if ~strcmp(fltRampUp_bkup,'0')
      |       set_param(gcb,'fltRampUp','0');
      |     end
      |   else
      |     tmps=num2str(fltRampUp);
      |     if ~strcmp(fltRampUp_bkup,tmps)
      |       set_param(gcb,'fltRampUp',tmps);
      |     end
      |   end
      |   if isnan(fltRampDown)
      |     if ~strcmp(fltRampDown_bkup,'0')
      |       set_param(gcb,'fltRampDown','0');
      |     end
      |   else
      |     tmps=num2str(fltRampDown);
      |     if ~strcmp(fltRampDown_bkup,tmps)
      |       set_param(gcb,'fltRampDown',tmps);
      |     end
      |   end
      | end
      mask Callback mechspeed:
      | autoCalcEn=get_param(gcb,'autoCalcEn');
      | if strcmp(autoCalcEn,'on')
      |   SampleTime=Simulink.data.evalinGlobal(bdroot,get_param(gcb,'SampleTime'));
      |   if (SampleTime==-1)
      |     SampleTime=str2double(get_param(gcb,'SampleTime_1'));
      |   end
      |   fltUmaxDivImax_bkup=get_param(gcb,'fltUmaxDivImax');
      |   fltLambdaW_bkup=get_param(gcb,'fltLambdaW');
      |   fltLambdaFW_bkup=get_param(gcb,'fltLambdaFW');
      |   fltPropGainQ_bkup=get_param(gcb,'fltPropGainQ');
      |   fltIntegGainQ_bkup=get_param(gcb,'fltIntegGainQ');
      |   fltLowerLimitQ_bkup=get_param(gcb,'fltLowerLimitQ');
      |   fltUpperLimitQ_bkup=get_param(gcb,'fltUpperLimitQ');
      |   fltPropGainFW_bkup=get_param(gcb,'fltPropGainFW');
      |   fltIntegGainFW_bkup=get_param(gcb,'fltIntegGainFW');
      |   fltLowerLimitFW_bkup=get_param(gcb,'fltLowerLimitFW');
      |   fltUpperLimitFW_bkup=get_param(gcb,'fltUpperLimitFW');
      |   fltRampUp_bkup=get_param(gcb,'fltRampUp');
      |   fltRampDown_bkup=get_param(gcb,'fltRampDown');
      |   wf0=Simulink.data.evalinGlobal(bdroot,get_param(gcb,'wf0'));
      |   wksi=Simulink.data.evalinGlobal(bdroot,get_param(gcb,'wksi'));
      |   J=Simulink.data.evalinGlobal(bdroot,get_param(gcb,'J'));
      |   Kt=Simulink.data.evalinGlobal(bdroot,get_param(gcb,'Kt'));
      |   lambdaW=Simulink.data.evalinGlobal(bdroot,get_param(gcb,'lambdaW'));
      |   lambdaFW=Simulink.data.evalinGlobal(bdroot,get_param(gcb,'lambdaFW'));
      |   Idmax=Simulink.data.evalinGlobal(bdroot,get_param(gcb,'Idmax'));
      |   imax=Simulink.data.evalinGlobal(bdroot,get_param(gcb,'imax'));
      |   udcbus=Simulink.data.evalinGlobal(bdroot,get_param(gcb,'udcbus'));
      |   ramprpm=Simulink.data.evalinGlobal(bdroot,get_param(gcb,'ramprpm'));
      |   mechspeed=Simulink.data.evalinGlobal(bdroot,get_param(gcb,'mechspeed'));
      |   polepairs=Simulink.data.evalinGlobal(bdroot,get_param(gcb,'polepairs'));
      |   if (wf0<=0)
      |     warning('Natural frequency f0 must be positive.');
      |   end
